simulink model "NN_v01"  (R2018b)
settings: Solver=VariableStepAuto  StartTime=0.0  StopTime=10.0  RelTol=1e-3
values from neighbouring files (symbols this model uses):
  B = 0.5    [Matlab_Newton_simulation_v01.m]    (also in NewtonMethod.m; NewtonMethod_2.m = 0.3; System_parameters.m = 0.3)
  b = f    (= 0.01)    [Matlab_Newton_simulation_v01.m]    (also in NewtonMethod.m; System_parameters.m)
  in_NN_data = [0 -100 -100 -100 -100 -100 -100 -100 -100 -100 -100 -100 ... (160801 elements, 401x401)]    [NN_IO_data.mat]    (also in NN_generate_input_data.m = con2seq(in_NN_data); NN_modelling_v02.m = con2seq(in_NN_data); NN_modelling_v03.m = con2seq(in_NN_data))
  l = 0.1    [Matlab_Newton_simulation_v01.m]    (also in NewtonMethod.m; NewtonMethod_2.m; System_parameters.m)
  m = 0.04    [Matlab_Newton_simulation_v01.m]    (also in NewtonMethod.m = 0.1; NewtonMethod_2.m; System_parameters.m)
  R = 1    [Matlab_Newton_simulation_v01.m]    (also in NewtonMethod.m; NewtonMethod_2.m = 0.1; System_parameters.m = 0.1)
libraries: neural x128
(part 5 of 5)

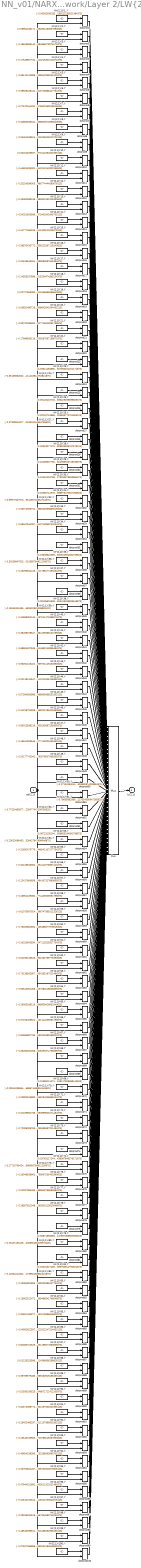
== system NN_v01/NARX Neural Network/Layer 2/LW{2,1} ==
  "ad{2,1}" : Inport  PortDimensions=10  SampleTime=1
      mask Display: e = 0.06;c1 = [120 230 180]/255;c2 = ([120 230 180]+0)/(256+128);c3 = ([120 230 180]+128)/(256+128);patch([0 1 1 0],[0 0 1 1],c1);patch([0 1 1 1-e 1-e 0+e],[0 0 1 1-e 0+e 0+e],c2);patch([0 0 1 1-e 0+e 0+e],[0 1 1 1-e 1-e 0+e],c3);plot([0 1 1 0 0],[0 0 1 1 0]);
  "IW{2,1}(1,:)'" : Constant  Value=[-0.00582930285020249842886652658080492983572185039520263671875;0.341294044267576091034044338812236674129962921142578125;0.275034396637413081077028209620038978755474090576171875;0.2474633161173106221664141912697232328355312347412109375;-1.50248270345251366819638860761187970638275146484375;0.7732400327116855098807945978478528559207916259765625;-0.463470385585337485423451653332449495792388916015625;-1.78313893365298614668290611007250845432281494140625;-0.8519246471113970375910184884560294449329376220703125;1.011244644169964512769865905283950269222259521484375]
      mask Display: e = 0.06;c1 = [120 150 230]/255;c2 = ([120 150 230]+0)/383;c3 = ([120 150 230]+128)/383;patch([0 1 1 0],[0 0 1 1],c1);patch([0 1 1 1-e 1-e 0+e],[0 0 1 1-e 0+e 0+e],c2);patch([0 0 1 1-e 0+e 0+e],[0 1 1 1-e 1-e 0+e],c3);plot([0 1 1 0 0],[0 0 1 1 0]);disp('weights');
  "IW{2,1}(10,:)'" : Constant  Value=[0.0020462983754603873871869001987988667679019272327423095703125;0.56448793796692864344066720150294713675975799560546875;1.50097031622448895404886570759117603302001953125;-0.43999986998791829062582792175817303359508514404296875;-2.436220494401638791970299280364997684955596923828125;0.90173545642475871897403294497053138911724090576171875;0.20243963357671435066009735237457789480686187744140625;0.359896850926928524305736800670274533331394195556640625;-0.9562162738582724585967298480682075023651123046875;1.2001988168349815300217642288771457970142364501953125]
      mask Display: e = 0.06;c1 = [120 150 230]/255;c2 = ([120 150 230]+0)/383;c3 = ([120 150 230]+128)/383;patch([0 1 1 0],[0 0 1 1],c1);patch([0 1 1 1-e 1-e 0+e],[0 0 1 1-e 0+e 0+e],c2);patch([0 0 1 1-e 0+e 0+e],[0 1 1 1-e 1-e 0+e],c3);plot([0 1 1 0 0],[0 0 1 1 0]);disp('weights');
  "IW{2,1}(100,:)'" : Constant  Value=[-0.07507286886552631821611925033721490763127803802490234375;0.59504324954741238951072546115028671920299530029296875;1.5961364935602364578670631090062670409679412841796875;-0.49363437154612432866684912369237281382083892822265625;-2.671162470519930831613919508527033030986785888671875;1.0123483498732077645598792514647357165813446044921875;0.236650285271016669330634840662241913378238677978515625;0.1698534154758429559617383119984879158437252044677734375;-1.2007351974579927311737037598504684865474700927734375;0.426723506364093230214251661891466937959194183349609375]
      mask Display: e = 0.06;c1 = [120 150 230]/255;c2 = ([120 150 230]+0)/383;c3 = ([120 150 230]+128)/383;patch([0 1 1 0],[0 0 1 1],c1);patch([0 1 1 1-e 1-e 0+e],[0 0 1 1-e 0+e 0+e],c2);patch([0 0 1 1-e 0+e 0+e],[0 1 1 1-e 1-e 0+e],c3);plot([0 1 1 0 0],[0 0 1 1 0]);disp('weights');
  "IW{2,1}(11,:)'" : Constant  Value=[-0.448513060024906928813237527720048092305660247802734375;0.64031830164589853549017561817890964448451995849609375;2.099861680687876486217646743170917034149169921875;-0.407344506580868459533206760170287452638149261474609375;-1.4883679183223523789791897797840647399425506591796875;1.4010738816362786618441305108717642724514007568359375;0.09498188052392357583197934900454129092395305633544921875;0.11685031296741331396926710795014514587819576263427734375;-1.1492554861913626407243782523437403142452239990234375;1.1105840548960890235008491799817420542240142822265625]
      mask Display: e = 0.06;c1 = [120 150 230]/255;c2 = ([120 150 230]+0)/383;c3 = ([120 150 230]+128)/383;patch([0 1 1 0],[0 0 1 1],c1);patch([0 1 1 1-e 1-e 0+e],[0 0 1 1-e 0+e 0+e],c2);patch([0 0 1 1-e 0+e 0+e],[0 1 1 1-e 1-e 0+e],c3);plot([0 1 1 0 0],[0 0 1 1 0]);disp('weights');
  "IW{2,1}(12,:)'" : Constant  Value=[-0.323245990037860642107858666349784471094608306884765625;0.702947047886376186198731375043280422687530517578125;2.15919372922789865043569079716689884662628173828125;-0.1613313202849812333372625516858533956110477447509765625;-2.691776450442475709934342376072891056537628173828125;1.3935502725959150183143719914369285106658935546875;-0.156722502399286034435732517522410489618778228759765625;-0.546597317678598759727037759148515760898590087890625;-0.0575394611420758927966545570598100312054157257080078125;0.2566683614467841767492473081802017986774444580078125]
      mask Display: e = 0.06;c1 = [120 150 230]/255;c2 = ([120 150 230]+0)/383;c3 = ([120 150 230]+128)/383;patch([0 1 1 0],[0 0 1 1],c1);patch([0 1 1 1-e 1-e 0+e],[0 0 1 1-e 0+e 0+e],c2);patch([0 0 1 1-e 0+e 0+e],[0 1 1 1-e 1-e 0+e],c3);plot([0 1 1 0 0],[0 0 1 1 0]);disp('weights');
  "IW{2,1}(13,:)'" : Constant  Value=[-0.45062389136594493965759511411306448280811309814453125;0.74707514561312782230828588581061922013759613037109375;2.534602836838535377950165639049373567104339599609375;0.681856533543756082593745304620824754238128662109375;-1.903748935623813309803153970278799533843994140625;1.486962257730305214664667801116593182086944580078125;-0.97748822795309264765961643206537701189517974853515625;-0.66163025511440742842950157864834181964397430419921875;-0.2757918190568944272200724299182184040546417236328125;0.3709896375713379601535280016832984983921051025390625]
      mask Display: e = 0.06;c1 = [120 150 230]/255;c2 = ([120 150 230]+0)/383;c3 = ([120 150 230]+128)/383;patch([0 1 1 0],[0 0 1 1],c1);patch([0 1 1 1-e 1-e 0+e],[0 0 1 1-e 0+e 0+e],c2);patch([0 0 1 1-e 0+e 0+e],[0 1 1 1-e 1-e 0+e],c3);plot([0 1 1 0 0],[0 0 1 1 0]);disp('weights');
  "IW{2,1}(14,:)'" : Constant  Value=[-0.54251603589707408925590925719006918370723724365234375;0.66743961741495472228535845715668983757495880126953125;2.25752081983530050734998440020717680454254150390625;-0.5193854735052190196853416637168265879154205322265625;-0.9760728597570194065013993167667649686336517333984375;1.5237519361875244694459752281545661389827728271484375;0.18414734508753072272924100616364739835262298583984375;-0.51378704789147111586800065197166986763477325439453125;-1.460284612501698386921589190023951232433319091796875;0.5274995341412360705390938164782710373401641845703125]
      mask Display: e = 0.06;c1 = [120 150 230]/255;c2 = ([120 150 230]+0)/383;c3 = ([120 150 230]+128)/383;patch([0 1 1 0],[0 0 1 1],c1);patch([0 1 1 1-e 1-e 0+e],[0 0 1 1-e 0+e 0+e],c2);patch([0 0 1 1-e 0+e 0+e],[0 1 1 1-e 1-e 0+e],c3);plot([0 1 1 0 0],[0 0 1 1 0]);disp('weights');
  "IW{2,1}(15,:)'" : Constant  Value=[-0.447774651064073492268136078564566560089588165283203125;0.791075818282777287748785965959541499614715576171875;2.658332437781770973828088244772516191005706787109375;0.19098785388139061236500992890796624124050140380859375;-2.357140652927365298552331296377815306186676025390625;1.6002796151954721270982417991035617887973785400390625;-0.533911807011674621747943092486821115016937255859375;-1.139783609828504129524162635789252817630767822265625;0.64540001022538107111614635869045741856098175048828125;0.231918187426728927835739568763528950512409210205078125]
      mask Display: e = 0.06;c1 = [120 150 230]/255;c2 = ([120 150 230]+0)/383;c3 = ([120 150 230]+128)/383;patch([0 1 1 0],[0 0 1 1],c1);patch([0 1 1 1-e 1-e 0+e],[0 0 1 1-e 0+e 0+e],c2);patch([0 0 1 1-e 0+e 0+e],[0 1 1 1-e 1-e 0+e],c3);plot([0 1 1 0 0],[0 0 1 1 0]);disp('weights');
  "IW{2,1}(16,:)'" : Constant  Value=[-0.368704337726813380360368910260149277746677398681640625;0.71983605028876151976646724506281316280364990234375;2.34431403126588211449643495143391191959381103515625;-0.284742382385777925701830781690659932792186737060546875;-2.320518919797865731169395075994543731212615966796875;1.45456918782064992257119229179807007312774658203125;-0.046608776255616470030052056472413823939859867095947265625;-0.44794291876033776045318290925933979451656341552734375;0.26754547078348134281355896746390499174594879150390625;0.8955736134500613676578950617113150656223297119140625]
      mask Display: e = 0.06;c1 = [120 150 230]/255;c2 = ([120 150 230]+0)/383;c3 = ([120 150 230]+128)/383;patch([0 1 1 0],[0 0 1 1],c1);patch([0 1 1 1-e 1-e 0+e],[0 0 1 1-e 0+e 0+e],c2);patch([0 0 1 1-e 0+e 0+e],[0 1 1 1-e 1-e 0+e],c3);plot([0 1 1 0 0],[0 0 1 1 0]);disp('weights');
  "IW{2,1}(17,:)'" : Constant  Value=[-0.316196432043710562442839773211744613945484161376953125;0.65170561350326738914162660876172594726085662841796875;2.052447913065332141258068077149800956249237060546875;0.1414451597873920551950988055978086777031421661376953125;-1.656287054632532118603194248862564563751220703125;1.2539456102076791399468902454827912151813507080078125;-0.41024093016196083727464838375453837215900421142578125;-0.305332211388109342475871699207345955073833465576171875;-1.38320146192491666425894436542876064777374267578125;0.34265345297769600474424578351317904889583587646484375]
      mask Display: e = 0.06;c1 = [120 150 230]/255;c2 = ([120 150 230]+0)/383;c3 = ([120 150 230]+128)/383;patch([0 1 1 0],[0 0 1 1],c1);patch([0 1 1 1-e 1-e 0+e],[0 0 1 1-e 0+e 0+e],c2);patch([0 0 1 1-e 0+e 0+e],[0 1 1 1-e 1-e 0+e],c3);plot([0 1 1 0 0],[0 0 1 1 0]);disp('weights');
  "IW{2,1}(18,:)'" : Constant  Value=[-0.1455533789674021971638495642764610238373279571533203125;0.6124068528724364579574057643185369670391082763671875;1.8468413066792230825541309968684799969196319580078125;0.2195780819216167356611180139225325547158718109130859375;-1.5780996737606607371873224110458977520465850830078125;1.0438697054205532399606681792647577822208404541015625;-0.452505406111580354977519391468376852571964263916015625;-0.257559752512215578423848683087271638214588165283203125;-1.2582096901281809575579018201096914708614349365234375;0.8091801339623978517323621417745016515254974365234375]
      mask Display: e = 0.06;c1 = [120 150 230]/255;c2 = ([120 150 230]+0)/383;c3 = ([120 150 230]+128)/383;patch([0 1 1 0],[0 0 1 1],c1);patch([0 1 1 1-e 1-e 0+e],[0 0 1 1-e 0+e 0+e],c2);patch([0 0 1 1-e 0+e 0+e],[0 1 1 1-e 1-e 0+e],c3);plot([0 1 1 0 0],[0 0 1 1 0]);disp('weights');
  "IW{2,1}(19,:)'" : Constant  Value=[0.0272765608292123602762746514827085775323212146759033203125;0.60751700312979561857673616032116115093231201171875;1.5496728878781473870418494698242284357547760009765625;-0.2376857676320399959113416343825520016252994537353515625;-3.088549185031914223742433023289777338504791259765625;0.92990955504973638046095629761111922562122344970703125;-0.00135475849347249720049102261754114806535653769969940185546875;-0.10569070740692888821232742202482768334448337554931640625;-0.959228755518120035361562258913181722164154052734375;0.017495673838348692330502132108449586667120456695556640625]
      mask Display: e = 0.06;c1 = [120 150 230]/255;c2 = ([120 150 230]+0)/383;c3 = ([120 150 230]+128)/383;patch([0 1 1 0],[0 0 1 1],c1);patch([0 1 1 1-e 1-e 0+e],[0 0 1 1-e 0+e 0+e],c2);patch([0 0 1 1-e 0+e 0+e],[0 1 1 1-e 1-e 0+e],c3);plot([0 1 1 0 0],[0 0 1 1 0]);disp('weights');
  "IW{2,1}(2,:)'" : Constant  Value=[0.05954166171467280277429523493992746807634830474853515625;0.40883309461008676688464902326813898980617523193359375;0.54706995308614458917162437501247040927410125732421875;-0.70577749899209096806629304410307668149471282958984375;-2.0501531346926782362061203457415103912353515625;0.79578752445065259468748308790964074432849884033203125;0.455298404531613964962843965622596442699432373046875;-1.261341483048185718729428117512725293636322021484375;-1.3307058361577859262325773670454509556293487548828125;0.351381921406758834791617118753492832183837890625]
      mask Display: e = 0.06;c1 = [120 150 230]/255;c2 = ([120 150 230]+0)/383;c3 = ([120 150 230]+128)/383;patch([0 1 1 0],[0 0 1 1],c1);patch([0 1 1 1-e 1-e 0+e],[0 0 1 1-e 0+e 0+e],c2);patch([0 0 1 1-e 0+e 0+e],[0 1 1 1-e 1-e 0+e],c3);plot([0 1 1 0 0],[0 0 1 1 0]);disp('weights');
  "IW{2,1}(20,:)'" : Constant  Value=[-0.038314807160081378045735078785583027638494968414306640625;0.64192842298741126239036702827434055507183074951171875;1.7730670440839084722739471544628031551837921142578125;-0.2070422965789282254700509611211600713431835174560546875;-2.049795488218523420442807037034071981906890869140625;1.05160185870840994226682596490718424320220947265625;-0.056829012384008115166267316453740932047367095947265625;-1.4674161260953708652010618607164360582828521728515625;-0.713738154031241744945646132691763341426849365234375;-0.280871218212835505045887884989497251808643341064453125]
      mask Display: e = 0.06;c1 = [120 150 230]/255;c2 = ([120 150 230]+0)/383;c3 = ([120 150 230]+128)/383;patch([0 1 1 0],[0 0 1 1],c1);patch([0 1 1 1-e 1-e 0+e],[0 0 1 1-e 0+e 0+e],c2);patch([0 0 1 1-e 0+e 0+e],[0 1 1 1-e 1-e 0+e],c3);plot([0 1 1 0 0],[0 0 1 1 0]);disp('weights');
  "IW{2,1}(21,:)'" : Constant  Value=[-0.59732069362601347695118647607159800827503204345703125;0.7944289114524234474146169304731301963329315185546875;2.771254282326547357939716675900854170322418212890625;-0.2278187864269799189909093684036633931100368499755859375;-2.350390468410268329790824282099492847919464111328125;1.769409008533941563001690155942924320697784423828125;-0.156797325798515074790628887058119289577007293701171875;-0.6081986540006287800252948727575130760669708251953125;0.9005540148021478064066513979923911392688751220703125;0.908050065992017874094699436682276427745819091796875]
      mask Display: e = 0.06;c1 = [120 150 230]/255;c2 = ([120 150 230]+0)/383;c3 = ([120 150 230]+128)/383;patch([0 1 1 0],[0 0 1 1],c1);patch([0 1 1 1-e 1-e 0+e],[0 0 1 1-e 0+e 0+e],c2);patch([0 0 1 1-e 0+e 0+e],[0 1 1 1-e 1-e 0+e],c3);plot([0 1 1 0 0],[0 0 1 1 0]);disp('weights');
  "IW{2,1}(22,:)'" : Constant  Value=[-0.1799665611847947044310558339930139482021331787109375;0.597358676332699456423824813100509345531463623046875;1.7143661042907727409811968755093403160572052001953125;-0.73930354885972360268198144694906659424304962158203125;-1.4961714010009259379074819662491790950298309326171875;1.122458137878769690587432705797255039215087890625;0.457656457228035329354298710313742049038410186767578125;-0.669106619974649152737811164115555584430694580078125;-1.6311188924677946232577596674673259258270263671875;0.219954413074346433187855609503458254039287567138671875]
      mask Display: e = 0.06;c1 = [120 150 230]/255;c2 = ([120 150 230]+0)/383;c3 = ([120 150 230]+128)/383;patch([0 1 1 0],[0 0 1 1],c1);patch([0 1 1 1-e 1-e 0+e],[0 0 1 1-e 0+e 0+e],c2);patch([0 0 1 1-e 0+e 0+e],[0 1 1 1-e 1-e 0+e],c3);plot([0 1 1 0 0],[0 0 1 1 0]);disp('weights');
  "IW{2,1}(23,:)'" : Constant  Value=[0.03514453865765392037712189221565495245158672332763671875;0.583844705291804100255603771074675023555755615234375;1.486426002621094699662762650405056774616241455078125;-0.90210579101266075152665280256769619882106781005859375;-2.997563508188325176462285526213236153125762939453125;0.94298906502310886335038730976521037518978118896484375;0.6341705941798434498224423805368132889270782470703125;0.1574250096667909326608736364505602978169918060302734375;-0.4923218586946191965836305826087482273578643798828125;0.90542674776050702245555612535099498927593231201171875]
      mask Display: e = 0.06;c1 = [120 150 230]/255;c2 = ([120 150 230]+0)/383;c3 = ([120 150 230]+128)/383;patch([0 1 1 0],[0 0 1 1],c1);patch([0 1 1 1-e 1-e 0+e],[0 0 1 1-e 0+e 0+e],c2);patch([0 0 1 1-e 0+e 0+e],[0 1 1 1-e 1-e 0+e],c3);plot([0 1 1 0 0],[0 0 1 1 0]);disp('weights');
  "IW{2,1}(24,:)'" : Constant  Value=[-0.35136664502954972899573249378590844571590423583984375;0.6736465513516909364710727459168992936611175537109375;2.144522192177507946553305373527109622955322265625;-0.5348072314147584993548889542580582201480865478515625;-1.8134291528864909803786531483638100326061248779296875;1.38047161618545288774839718826115131378173828125;0.21260601550874402843049892908311448991298675537109375;-0.5304234087346137993534966881270520389080047607421875;-0.574433193811335396361528182751499116420745849609375;0.67345838441960104159278444058145396411418914794921875]
      mask Display: e = 0.06;c1 = [120 150 230]/255;c2 = ([120 150 230]+0)/383;c3 = ([120 150 230]+128)/383;patch([0 1 1 0],[0 0 1 1],c1);patch([0 1 1 1-e 1-e 0+e],[0 0 1 1-e 0+e 0+e],c2);patch([0 0 1 1-e 0+e 0+e],[0 1 1 1-e 1-e 0+e],c3);plot([0 1 1 0 0],[0 0 1 1 0]);disp('weights');
  "IW{2,1}(25,:)'" : Constant  Value=[0.05149415733482787249641887683537788689136505126953125;0.55009804320874489125259287902736105024814605712890625;1.4573734074988748954382344891200773417949676513671875;0.203985369914554570680564893336850218474864959716796875;-2.108439519484554214301397223607636988162994384765625;0.7713724398957200190096727965283207595348358154296875;-0.38913427522632348942721591811277903616428375244140625;0.40356097259732670590182124215061776340007781982421875;-1.686695031530128563446169209782965481281280517578125;0.89980821268971344917275700936443172395229339599609375]
      mask Display: e = 0.06;c1 = [120 150 230]/255;c2 = ([120 150 230]+0)/383;c3 = ([120 150 230]+128)/383;patch([0 1 1 0],[0 0 1 1],c1);patch([0 1 1 1-e 1-e 0+e],[0 0 1 1-e 0+e 0+e],c2);patch([0 0 1 1-e 0+e 0+e],[0 1 1 1-e 1-e 0+e],c3);plot([0 1 1 0 0],[0 0 1 1 0]);disp('weights');
  "IW{2,1}(26,:)'" : Constant  Value=[0.02204713886760389929264647435047663748264312744140625;0.5921585247554281838944234550581313669681549072265625;1.55519918105156396137545016244985163211822509765625;-0.51973881437109403780283400919870473444461822509765625;-2.912447784998210220663850122946314513683319091796875;0.93575628387550702225183840710087679326534271240234375;0.268635001612249457725312140610185451805591583251953125;0.2139320565909990923270100893205380998551845550537109375;-0.5458971643579728638684400721103884279727935791015625;0.93073309088335609562392392035690136253833770751953125]
      mask Display: e = 0.06;c1 = [120 150 230]/255;c2 = ([120 150 230]+0)/383;c3 = ([120 150 230]+128)/383;patch([0 1 1 0],[0 0 1 1],c1);patch([0 1 1 1-e 1-e 0+e],[0 0 1 1-e 0+e 0+e],c2);patch([0 0 1 1-e 0+e 0+e],[0 1 1 1-e 1-e 0+e],c3);plot([0 1 1 0 0],[0 0 1 1 0]);disp('weights');
  "IW{2,1}(27,:)'" : Constant  Value=[-0.37908624877066599001551594483316875994205474853515625;0.7418677921218022053295726436772383749485015869140625;2.443837843676642140877675046795047819614410400390625;-0.02623926447862567901125885327928699553012847900390625;-2.2303123439129013405590740148909389972686767578125;1.4856482550534242381701233171042986214160919189453125;-0.303941770708726632932439315482042729854583740234375;-0.82184113198571473457576530563528649508953094482421875;0.485827492873038779830352495991974137723445892333984375;0.72913166625223502226305072326795198023319244384765625]
      mask Display: e = 0.06;c1 = [120 150 230]/255;c2 = ([120 150 230]+0)/383;c3 = ([120 150 230]+128)/383;patch([0 1 1 0],[0 0 1 1],c1);patch([0 1 1 1-e 1-e 0+e],[0 0 1 1-e 0+e 0+e],c2);patch([0 0 1 1-e 0+e 0+e],[0 1 1 1-e 1-e 0+e],c3);plot([0 1 1 0 0],[0 0 1 1 0]);disp('weights');
  "IW{2,1}(28,:)'" : Constant  Value=[0.0262307747004455575623449448130486416630446910858154296875;0.6141526444488019098599806966376490890979766845703125;1.68407366789876089541166948038153350353240966796875;0.396007677131411828241880357381887733936309814453125;-2.224396987240094603066609124653041362762451171875;0.89300425378741821180739179908414371311664581298828125;-0.6041927337275698750573837969568558037281036376953125;-0.586160540594302670314164060982875525951385498046875;-1.0496445142758663582327471885946579277515411376953125;0.1955911512259201068264502509919111616909503936767578125]
      mask Display: e = 0.06;c1 = [120 150 230]/255;c2 = ([120 150 230]+0)/383;c3 = ([120 150 230]+128)/383;patch([0 1 1 0],[0 0 1 1],c1);patch([0 1 1 1-e 1-e 0+e],[0 0 1 1-e 0+e 0+e],c2);patch([0 0 1 1-e 0+e 0+e],[0 1 1 1-e 1-e 0+e],c3);plot([0 1 1 0 0],[0 0 1 1 0]);disp('weights');
  "IW{2,1}(29,:)'" : Constant  Value=[0.0246853775513488395143557596611572080291807651519775390625;0.57664087857391665981054984513320960104465484619140625;1.519319484599648273359662198345176875591278076171875;-0.414640620269337734082881752328830771148204803466796875;-2.36036201032834380697522647096775472164154052734375;0.8965136872108658838698147519608028233051300048828125;0.177479815810386798435871469337143935263156890869140625;-0.0696335087218894199789787080590031109750270843505859375;-1.038098982722849061843817253247834742069244384765625;0.74747558926703472348407331082853488624095916748046875]
      mask Display: e = 0.06;c1 = [120 150 230]/255;c2 = ([120 150 230]+0)/383;c3 = ([120 150 230]+128)/383;patch([0 1 1 0],[0 0 1 1],c1);patch([0 1 1 1-e 1-e 0+e],[0 0 1 1-e 0+e 0+e],c2);patch([0 0 1 1-e 0+e 0+e],[0 1 1 1-e 1-e 0+e],c3);plot([0 1 1 0 0],[0 0 1 1 0]);disp('weights');
  "IW{2,1}(3,:)'" : Constant  Value=[-0.1684585614083785320982400435241288505494594573974609375;0.48589007836087583225292974020703695714473724365234375;1.1686058202574383102501087705604732036590576171875;-0.0581777076386999769663788129037129692733287811279296875;-1.262969470679580208383185890852473676204681396484375;1.009868185502584392310154726146720349788665771484375;-0.191550045020977333098954886736464686691761016845703125;-0.8789087611980193059935118071734905242919921875;-1.4777892930254401537837338764802552759647369384765625;0.82183474981515203250381773614208213984966278076171875]
      mask Display: e = 0.06;c1 = [120 150 230]/255;c2 = ([120 150 230]+0)/383;c3 = ([120 150 230]+128)/383;patch([0 1 1 0],[0 0 1 1],c1);patch([0 1 1 1-e 1-e 0+e],[0 0 1 1-e 0+e 0+e],c2);patch([0 0 1 1-e 0+e 0+e],[0 1 1 1-e 1-e 0+e],c3);plot([0 1 1 0 0],[0 0 1 1 0]);disp('weights');
  "IW{2,1}(30,:)'" : Constant  Value=[0.1525421876865361292541223292573704384267330169677734375;0.59280217846434168915692453083465807139873504638671875;1.5103998560570150999637917266227304935455322265625;0.6179532744324938153823723041568882763385772705078125;-2.27436947201279071606450088438577950000762939453125;0.73383641375792552086210207562544383108615875244140625;-0.79185101288714199174734176267520524561405181884765625;-0.78250730160382298006283008362515829503536224365234375;-1.3421010523912026979331812981399707496166229248046875;-0.170860963215741123999436013036756776273250579833984375]
      mask Display: e = 0.06;c1 = [120 150 230]/255;c2 = ([120 150 230]+0)/383;c3 = ([120 150 230]+128)/383;patch([0 1 1 0],[0 0 1 1],c1);patch([0 1 1 1-e 1-e 0+e],[0 0 1 1-e 0+e 0+e],c2);patch([0 0 1 1-e 0+e 0+e],[0 1 1 1-e 1-e 0+e],c3);plot([0 1 1 0 0],[0 0 1 1 0]);disp('weights');
  "IW{2,1}(31,:)'" : Constant  Value=[0.25380712576948349923355863211327232420444488525390625;0.492216462292187573179802484446554444730281829833984375;0.99693922666631429319039625625009648501873016357421875;-0.49533921863121566087073688322561793029308319091796875;-2.790527644025747378009327803738415241241455078125;0.56383871163692311778703469826723448932170867919921875;0.31609849703952985766619576679659076035022735595703125;0.50949914899270487556037778631434775888919830322265625;-1.9496983918952286440884336116141639649868011474609375;0.50011526375033188429597430513240396976470947265625]
      mask Display: e = 0.06;c1 = [120 150 230]/255;c2 = ([120 150 230]+0)/383;c3 = ([120 150 230]+128)/383;patch([0 1 1 0],[0 0 1 1],c1);patch([0 1 1 1-e 1-e 0+e],[0 0 1 1-e 0+e 0+e],c2);patch([0 0 1 1-e 0+e 0+e],[0 1 1 1-e 1-e 0+e],c3);plot([0 1 1 0 0],[0 0 1 1 0]);disp('weights');
  "IW{2,1}(32,:)'" : Constant  Value=[-0.59977927573484135503889547180733643472194671630859375;0.78607459639563870279488355663488619029521942138671875;2.72389386341507577782294902135618031024932861328125;-0.373262242287550394248540897024213336408138275146484375;-2.49918566630663452343696917523629963397979736328125;1.77057144387650833294856056454591453075408935546875;-0.0165541406353492855096920521873471443541347980499267578125;-0.40925534192587742499114256133907474577426910400390625;0.8975452209878096443418371563893742859363555908203125;0.9980060058792241672875888980343006551265716552734375]
      mask Display: e = 0.06;c1 = [120 150 230]/255;c2 = ([120 150 230]+0)/383;c3 = ([120 150 230]+128)/383;patch([0 1 1 0],[0 0 1 1],c1);patch([0 1 1 1-e 1-e 0+e],[0 0 1 1-e 0+e 0+e],c2);patch([0 0 1 1-e 0+e 0+e],[0 1 1 1-e 1-e 0+e],c3);plot([0 1 1 0 0],[0 0 1 1 0]);disp('weights');
  "IW{2,1}(33,:)'" : Constant  Value=[-0.05374356701386216739191326041691354475915431976318359375;0.60138254176158145725139547721482813358306884765625;1.599503658211905321451240524766035377979278564453125;-0.8636852631541216407384808917413465678691864013671875;-2.845568136452600871422191630699671804904937744140625;1.0405825744174703739730603047064505517482757568359375;0.58290688850284488875530541918124072253704071044921875;0.051528965566472302584077880283075501210987567901611328125;-0.66103580577425147257741855355561710894107818603515625;0.66779080122559675292137626456678844988346099853515625]
      mask Display: e = 0.06;c1 = [120 150 230]/255;c2 = ([120 150 230]+0)/383;c3 = ([120 150 230]+128)/383;patch([0 1 1 0],[0 0 1 1],c1);patch([0 1 1 1-e 1-e 0+e],[0 0 1 1-e 0+e 0+e],c2);patch([0 0 1 1-e 0+e 0+e],[0 1 1 1-e 1-e 0+e],c3);plot([0 1 1 0 0],[0 0 1 1 0]);disp('weights');
  "IW{2,1}(34,:)'" : Constant  Value=[-0.581678440979031652346975533873774111270904541015625;0.81326669444152577259643521756515838205814361572265625;2.89315911107999834683823792147450149059295654296875;0.70491023718167389322530880235717631876468658447265625;-2.18278968945419915570482771727256476879119873046875;1.7147670503171494882366232559434138238430023193359375;-1.045237944023320597608517346088774502277374267578125;-0.70802493541687494538194869164726696908473968505859375;0.880677613510830070708834682591259479522705078125;0.84463766908679482892097212243243120610713958740234375]
      mask Display: e = 0.06;c1 = [120 150 230]/255;c2 = ([120 150 230]+0)/383;c3 = ([120 150 230]+128)/383;patch([0 1 1 0],[0 0 1 1],c1);patch([0 1 1 1-e 1-e 0+e],[0 0 1 1-e 0+e 0+e],c2);patch([0 0 1 1-e 0+e 0+e],[0 1 1 1-e 1-e 0+e],c3);plot([0 1 1 0 0],[0 0 1 1 0]);disp('weights');
  "IW{2,1}(35,:)'" : Constant  Value=[0.196066220897142706736104855735902674496173858642578125;0.56114967567245077617599235964007675647735595703125;1.3132272740157155954676682085846550762653350830078125;-0.190190351808331492566850329239969141781330108642578125;-3.4050286399046942875656895921565592288970947265625;0.711621044678856673471045723999850451946258544921875;-0.01169746299349863453975739702173086698167026042938232421875;0.53162953097797494006471197280916385352611541748046875;-0.6906821766335207168907572850002907216548919677734375;0.8527130315578423935818364043370820581912994384765625]
      mask Display: e = 0.06;c1 = [120 150 230]/255;c2 = ([120 150 230]+0)/383;c3 = ([120 150 230]+128)/383;patch([0 1 1 0],[0 0 1 1],c1);patch([0 1 1 1-e 1-e 0+e],[0 0 1 1-e 0+e 0+e],c2);patch([0 0 1 1-e 0+e 0+e],[0 1 1 1-e 1-e 0+e],c3);plot([0 1 1 0 0],[0 0 1 1 0]);disp('weights');
  "IW{2,1}(36,:)'" : Constant  Value=[-0.30238847823709935624947320320643484592437744140625;0.63809581334946396946605773337068967521190643310546875;1.93841310136525013518848936655558645725250244140625;-0.76799610669453122202554595787660218775272369384765625;-1.790601099870265944247194056515581905841827392578125;1.2946912691900547276446786781889386475086212158203125;0.455166148167682471648021191867883317172527313232421875;-0.449030326835419713038533018334419466555118560791015625;-1.1676394023242508968252195700188167393207550048828125;0.383807058733641459635776982395327650010585784912109375]
      mask Display: e = 0.06;c1 = [120 150 230]/255;c2 = ([120 150 230]+0)/383;c3 = ([120 150 230]+128)/383;patch([0 1 1 0],[0 0 1 1],c1);patch([0 1 1 1-e 1-e 0+e],[0 0 1 1-e 0+e 0+e],c2);patch([0 0 1 1-e 0+e 0+e],[0 1 1 1-e 1-e 0+e],c3);plot([0 1 1 0 0],[0 0 1 1 0]);disp('weights');
  "IW{2,1}(37,:)'" : Constant  Value=[-0.452936344163830550968441457371227443218231201171875;0.76433820653682549295382386844721622765064239501953125;2.56830362490622832183362334035336971282958984375;0.5183817105699082272707300944603048264980316162109375;-1.8382729426133825878508787354803644120693206787109375;1.5372946831195355432697624564752914011478424072265625;-0.83324123394107785234297125498414970934391021728515625;-1.2789096058712516867927888597478158771991729736328125;-0.106021597656944133181156075806939043104648590087890625;-0.054355271524427505036580754449460073374211788177490234375]
      mask Display: e = 0.06;c1 = [120 150 230]/255;c2 = ([120 150 230]+0)/383;c3 = ([120 150 230]+128)/383;patch([0 1 1 0],[0 0 1 1],c1);patch([0 1 1 1-e 1-e 0+e],[0 0 1 1-e 0+e 0+e],c2);patch([0 0 1 1-e 0+e 0+e],[0 1 1 1-e 1-e 0+e],c3);plot([0 1 1 0 0],[0 0 1 1 0]);disp('weights');
  "IW{2,1}(38,:)'" : Constant  Value=[0.09136601508625417922271338966311304830014705657958984375;0.62253057715237625213688943404122255742549896240234375;1.627047130871312585753685198142193257808685302734375;0.176907776487810475263273701784783042967319488525390625;-2.82675092583253739775273061241023242473602294921875;0.87596723158291622812754440019489265978336334228515625;-0.396760044760268326680119344018748961389064788818359375;-0.60181119810399430480885030192439444363117218017578125;-0.53741128759564638084356147373910062015056610107421875;0.1372008230337089240702397319182637147605419158935546875]
      mask Display: e = 0.06;c1 = [120 150 230]/255;c2 = ([120 150 230]+0)/383;c3 = ([120 150 230]+128)/383;patch([0 1 1 0],[0 0 1 1],c1);patch([0 1 1 1-e 1-e 0+e],[0 0 1 1-e 0+e 0+e],c2);patch([0 0 1 1-e 0+e 0+e],[0 1 1 1-e 1-e 0+e],c3);plot([0 1 1 0 0],[0 0 1 1 0]);disp('weights');
  "IW{2,1}(39,:)'" : Constant  Value=[-0.1834530433555252304511640204509603790938854217529296875;0.59972841849818703252594787045381963253021240234375;1.80972193123266134051618792000226676464080810546875;-0.214511595761017748174026564811356365680694580078125;-1.818294281749900154210308755864389240741729736328125;1.0839633537532911145007119557703845202922821044921875;-0.038703040293351233247509668444763519801199436187744140625;0.31497073227985061816269762857700698077678680419921875;-1.217905982251902496926732055726461112499237060546875;1.219166080770367699415146489627659320831298828125]
      mask Display: e = 0.06;c1 = [120 150 230]/255;c2 = ([120 150 230]+0)/383;c3 = ([120 150 230]+128)/383;patch([0 1 1 0],[0 0 1 1],c1);patch([0 1 1 1-e 1-e 0+e],[0 0 1 1-e 0+e 0+e],c2);patch([0 0 1 1-e 0+e 0+e],[0 1 1 1-e 1-e 0+e],c3);plot([0 1 1 0 0],[0 0 1 1 0]);disp('weights');
  "IW{2,1}(4,:)'" : Constant  Value=[-0.1764985773415378711437284664498292841017246246337890625;0.550065938829558565004163028788752853870391845703125;1.400052168430072629945470907841809093952178955078125;0.132046705074750747588296917456318624317646026611328125;-1.7551038520745418924917657932383008301258087158203125;1.1042013956640885918858430159161798655986785888671875;-0.398070213018517471414980946065043099224567413330078125;-1.2779459978482663462528989839483983814716339111328125;-0.74348434077020153498693844085210002958774566650390625;0.43747499192806316159476409666240215301513671875]
      mask Display: e = 0.06;c1 = [120 150 230]/255;c2 = ([120 150 230]+0)/383;c3 = ([120 150 230]+128)/383;patch([0 1 1 0],[0 0 1 1],c1);patch([0 1 1 1-e 1-e 0+e],[0 0 1 1-e 0+e 0+e],c2);patch([0 0 1 1-e 0+e 0+e],[0 1 1 1-e 1-e 0+e],c3);plot([0 1 1 0 0],[0 0 1 1 0]);disp('weights');
  "IW{2,1}(40,:)'" : Constant  Value=[-0.34868091134588075075129154356545768678188323974609375;0.71163976165356579439702500167186371982097625732421875;2.25914385259164962604927495704032480716705322265625;0.1577562521924193161826366349487216211855411529541015625;-1.915798113589740836459895945154130458831787109375;1.38767243601959489041064443881623446941375732421875;-0.457821625679664945263169784084311686456203460693359375;-1.08565360321842252488977464963681995868682861328125;-0.682343662616461177350402067531831562519073486328125;-0.212814032725580914995333614569972269237041473388671875]
      mask Display: e = 0.06;c1 = [120 150 230]/255;c2 = ([120 150 230]+0)/383;c3 = ([120 150 230]+128)/383;patch([0 1 1 0],[0 0 1 1],c1);patch([0 1 1 1-e 1-e 0+e],[0 0 1 1-e 0+e 0+e],c2);patch([0 0 1 1-e 0+e 0+e],[0 1 1 1-e 1-e 0+e],c3);plot([0 1 1 0 0],[0 0 1 1 0]);disp('weights');
  "IW{2,1}(41,:)'" : Constant  Value=[-0.384693786478920163318662162055261433124542236328125;0.670405982836017155790386823355220258235931396484375;2.233547800532729610267779207788407802581787109375;0.29885623813081096944443970642169006168842315673828125;-1.1614848768459038463873866930953226983547210693359375;1.328849739927486783841459327959455549716949462890625;-0.57382634252319297818445420489297248423099517822265625;-0.50487318014105142527370162497390992939472198486328125;-1.2223651496305525387953139215824194252490997314453125;0.63080717880939707331577892546192742884159088134765625]
      mask Display: e = 0.06;c1 = [120 150 230]/255;c2 = ([120 150 230]+0)/383;c3 = ([120 150 230]+128)/383;patch([0 1 1 0],[0 0 1 1],c1);patch([0 1 1 1-e 1-e 0+e],[0 0 1 1-e 0+e 0+e],c2);patch([0 0 1 1-e 0+e 0+e],[0 1 1 1-e 1-e 0+e],c3);plot([0 1 1 0 0],[0 0 1 1 0]);disp('weights');
  "IW{2,1}(42,:)'" : Constant  Value=[-0.68954337845844893006841402893769554793834686279296875;0.76156028935077468844383474788628518581390380859375;2.733377962340927780360289034433662891387939453125;-0.3307189584512639779489973079762421548366546630859375;-1.767964860054358045005074018263258039951324462890625;1.7925680718506515898269526587682776153087615966796875;-0.05147072696549311043856533842699718661606311798095703125;-0.206982244610009080698631578343338333070278167724609375;0.11909077605025293611351600020498153753578662872314453125;1.152960876683140067910926518379710614681243896484375]
      mask Display: e = 0.06;c1 = [120 150 230]/255;c2 = ([120 150 230]+0)/383;c3 = ([120 150 230]+128)/383;patch([0 1 1 0],[0 0 1 1],c1);patch([0 1 1 1-e 1-e 0+e],[0 0 1 1-e 0+e 0+e],c2);patch([0 0 1 1-e 0+e 0+e],[0 1 1 1-e 1-e 0+e],c3);plot([0 1 1 0 0],[0 0 1 1 0]);disp('weights');
  "IW{2,1}(43,:)'" : Constant  Value=[-0.5929121540110366961329191326512955129146575927734375;0.70738919924875631739524806107510812580585479736328125;2.376005332543118075960819624015130102634429931640625;-0.76158579503022927337241299028391949832439422607421875;-2.10889938205355065292678773403167724609375;1.6506375691719892273567893425934016704559326171875;0.3913239221352433627743039323831908404827117919921875;0.10400934437467583559833173012521001510322093963623046875;-0.64661658623874285201083011997980065643787384033203125;0.69885919020168041360108190929167903959751129150390625]
      mask Display: e = 0.06;c1 = [120 150 230]/255;c2 = ([120 150 230]+0)/383;c3 = ([120 150 230]+128)/383;patch([0 1 1 0],[0 0 1 1],c1);patch([0 1 1 1-e 1-e 0+e],[0 0 1 1-e 0+e 0+e],c2);patch([0 0 1 1-e 0+e 0+e],[0 1 1 1-e 1-e 0+e],c3);plot([0 1 1 0 0],[0 0 1 1 0]);disp('weights');
  "IW{2,1}(44,:)'" : Constant  Value=[-0.0211814254701263859903548336660605855286121368408203125;0.5988864812756748978728182919439859688282012939453125;1.6910868744764149251835760878748260438442230224609375;0.40914415135783899213350878198980353772640228271484375;-1.895921791759112462472103288746438920497894287109375;0.9007222790673903300984193265321664512157440185546875;-0.61261974959761233971988758639781735837459564208984375;-0.301489605795037307611750065916567109525203704833984375;-1.3838127391879766481253000165452249348163604736328125;0.47532435357247226903609771397896111011505126953125]
      mask Display: e = 0.06;c1 = [120 150 230]/255;c2 = ([120 150 230]+0)/383;c3 = ([120 150 230]+128)/383;patch([0 1 1 0],[0 0 1 1],c1);patch([0 1 1 1-e 1-e 0+e],[0 0 1 1-e 0+e 0+e],c2);patch([0 0 1 1-e 0+e 0+e],[0 1 1 1-e 1-e 0+e],c3);plot([0 1 1 0 0],[0 0 1 1 0]);disp('weights');
  "IW{2,1}(45,:)'" : Constant  Value=[-0.57394830886734815589278468905831687152385711669921875;0.7758353840895348962902744460734538733959197998046875;2.729870216737170895981989815481938421726226806640625;0.486636550182550975396367221037507988512516021728515625;-1.73848539994374018391454228549264371395111083984375;1.6575732242535277105588420454296283423900604248046875;-0.819449929931143739025856120861135423183441162109375;-0.79445874364760593611123340451740659773349761962890625;0.062040531257998583758439536950390902347862720489501953125;0.5443755628008635216730226602521724998950958251953125]
      mask Display: e = 0.06;c1 = [120 150 230]/255;c2 = ([120 150 230]+0)/383;c3 = ([120 150 230]+128)/383;patch([0 1 1 0],[0 0 1 1],c1);patch([0 1 1 1-e 1-e 0+e],[0 0 1 1-e 0+e 0+e],c2);patch([0 0 1 1-e 0+e 0+e],[0 1 1 1-e 1-e 0+e],c3);plot([0 1 1 0 0],[0 0 1 1 0]);disp('weights');
  "IW{2,1}(46,:)'" : Constant  Value=[-0.41218791808006749466386509084259159862995147705078125;0.68294697094525858016567099184612743556499481201171875;2.1812169635464524475310099660418927669525146484375;-0.3122138439025423650718948920257389545440673828125;-2.3919144846367839107870167936198413372039794921875;1.4249365798424140638900325939175672829151153564453125;-0.005641744161312560283672024041834447416476905345916748046875;0.17410184172223341914076399916666559875011444091796875;-0.673316563070028184512239022296853363513946533203125;0.65772099647677573219795021941536106169223785400390625]
      mask Display: e = 0.06;c1 = [120 150 230]/255;c2 = ([120 150 230]+0)/383;c3 = ([120 150 230]+128)/383;patch([0 1 1 0],[0 0 1 1],c1);patch([0 1 1 1-e 1-e 0+e],[0 0 1 1-e 0+e 0+e],c2);patch([0 0 1 1-e 0+e 0+e],[0 1 1 1-e 1-e 0+e],c3);plot([0 1 1 0 0],[0 0 1 1 0]);disp('weights');
  "IW{2,1}(47,:)'" : Constant  Value=[-0.6601283821964922804426123548182658851146697998046875;0.71682210829467063462061560130678117275238037109375;2.507777607825319332590652265935204923152923583984375;-0.4691640106248977648562004105770029127597808837890625;-0.84098642960201963614252917977864854037761688232421875;1.6957724169771568600850741859176196157932281494140625;0.10582480693325056753106849782852805219590663909912109375;-0.97280418442449756444290187573642469942569732666015625;-1.334943670733434561981312072020955383777618408203125;0.078976933807087090766430037547252140939235687255859375]
      mask Display: e = 0.06;c1 = [120 150 230]/255;c2 = ([120 150 230]+0)/383;c3 = ([120 150 230]+128)/383;patch([0 1 1 0],[0 0 1 1],c1);patch([0 1 1 1-e 1-e 0+e],[0 0 1 1-e 0+e 0+e],c2);patch([0 0 1 1-e 0+e 0+e],[0 1 1 1-e 1-e 0+e],c3);plot([0 1 1 0 0],[0 0 1 1 0]);disp('weights');
  "IW{2,1}(48,:)'" : Constant  Value=[-0.456419298439418030799430425759055651724338531494140625;0.72313861048824179533767164684832096099853515625;2.40986742146247134854775140411220490932464599609375;0.0214512669821436165185080113815274671651422977447509765625;-1.19680450750258149383853378822095692157745361328125;1.5060527348488850218899415267514996230602264404296875;-0.34414919860015469321723458051565103232860565185546875;-1.482143618281361430177867077873088419437408447265625;-0.82798638096933807606347954788361676037311553955078125;-0.1802135218681593376022220809318241663277149200439453125]
      mask Display: e = 0.06;c1 = [120 150 230]/255;c2 = ([120 150 230]+0)/383;c3 = ([120 150 230]+128)/383;patch([0 1 1 0],[0 0 1 1],c1);patch([0 1 1 1-e 1-e 0+e],[0 0 1 1-e 0+e 0+e],c2);patch([0 0 1 1-e 0+e 0+e],[0 1 1 1-e 1-e 0+e],c3);plot([0 1 1 0 0],[0 0 1 1 0]);disp('weights');
  "IW{2,1}(49,:)'" : Constant  Value=[-0.201777420421350106582991656978265382349491119384765625;0.62191621841690125638280051134643144905567169189453125;1.8119283917398167904622141577419824898242950439453125;-0.5227232263910142062712793631362728774547576904296875;-2.439458773395342117140671689412556588649749755859375;1.1650190345772750699637754223658703267574310302734375;0.23989752362414018538316895501338876783847808837890625;0.205855921277374231959100825406494550406932830810546875;-0.9529096895648516696297747330390848219394683837890625;0.73215887561226222768340221591643057763576507568359375]
      mask Display: e = 0.06;c1 = [120 150 230]/255;c2 = ([120 150 230]+0)/383;c3 = ([120 150 230]+128)/383;patch([0 1 1 0],[0 0 1 1],c1);patch([0 1 1 1-e 1-e 0+e],[0 0 1 1-e 0+e 0+e],c2);patch([0 0 1 1-e 0+e 0+e],[0 1 1 1-e 1-e 0+e],c3);plot([0 1 1 0 0],[0 0 1 1 0]);disp('weights');
  "IW{2,1}(5,:)'" : Constant  Value=[-0.361104428885895167855579757087980397045612335205078125;0.63294787419499787262111567542888224124908447265625;2.070132619536046991726152555202133953571319580078125;0.420864372235277894862548464516294188797473907470703125;-1.485100440670633847872750266105867922306060791015625;1.25189228417873099630241995328105986118316650390625;-0.6766670609109386447244105511344969272613525390625;0.262109587209254535355995585632626898586750030517578125;-1.23739336927696097490070314961485564708709716796875;1.2100048860681276163830943914945237338542938232421875]
      mask Display: e = 0.06;c1 = [120 150 230]/255;c2 = ([120 150 230]+0)/383;c3 = ([120 150 230]+128)/383;patch([0 1 1 0],[0 0 1 1],c1);patch([0 1 1 1-e 1-e 0+e],[0 0 1 1-e 0+e 0+e],c2);patch([0 0 1 1-e 0+e 0+e],[0 1 1 1-e 1-e 0+e],c3);plot([0 1 1 0 0],[0 0 1 1 0]);disp('weights');
  "IW{2,1}(50,:)'" : Constant  Value=[-0.1710439451457241577525536513348924927413463592529296875;0.6582236969091852518687346673686988651752471923828125;2.011306021194341209223921396187506616115570068359375;0.38087735787934651199293512036092579364776611328125;-2.826802661426973894975844814325682818889617919921875;1.132059008564136437513525379472412168979644775390625;-0.6287175867037755327970671714865602552890777587890625;0.559666047608690764292305175331421196460723876953125;-0.154249598879783234028906235835165716707706451416015625;1.31421098450051854200637535541318356990814208984375]
      mask Display: e = 0.06;c1 = [120 150 230]/255;c2 = ([120 150 230]+0)/383;c3 = ([120 150 230]+128)/383;patch([0 1 1 0],[0 0 1 1],c1);patch([0 1 1 1-e 1-e 0+e],[0 0 1 1-e 0+e 0+e],c2);patch([0 0 1 1-e 0+e 0+e],[0 1 1 1-e 1-e 0+e],c3);plot([0 1 1 0 0],[0 0 1 1 0]);disp('weights');
  "IW{2,1}(51,:)'" : Constant  Value=[-0.79655882956646217873952764421119354665279388427734375;0.78415898119855464987182358527206815779209136962890625;2.91708511729693942271524065290577709674835205078125;-0.0223287146166207713104956411598323029465973377227783203125;-1.2530913987062886061352173783234320580959320068359375;1.8915671695448548206286432105116546154022216796875;-0.3616281011241284648605187612702138721942901611328125;-0.494062157839597226871575230688904412090778350830078125;-0.156785330838478065285102047710097394883632659912109375;0.926573513474272747458826415822841227054595947265625]
      mask Display: e = 0.06;c1 = [120 150 230]/255;c2 = ([120 150 230]+0)/383;c3 = ([120 150 230]+128)/383;patch([0 1 1 0],[0 0 1 1],c1);patch([0 1 1 1-e 1-e 0+e],[0 0 1 1-e 0+e 0+e],c2);patch([0 0 1 1-e 0+e 0+e],[0 1 1 1-e 1-e 0+e],c3);plot([0 1 1 0 0],[0 0 1 1 0]);disp('weights');
  "IW{2,1}(52,:)'" : Constant  Value=[-0.77520483877998980215551227956893853843212127685546875;0.77360216709961016068319850091938860714435577392578125;2.84526158862346445488356039277277886867523193359375;-0.124298281629053153363173578327405266463756561279296875;-1.3712902310571788433435358456335961818695068359375;1.8635474347286684615454532831790857017040252685546875;-0.258231915472281470247395418482483364641666412353515625;-0.38754152309492628791787183217820711433887481689453125;-0.25448599483401668219784141911077313125133514404296875;0.8858499832048656319472001996473409235477447509765625]
      mask Display: e = 0.06;c1 = [120 150 230]/255;c2 = ([120 150 230]+0)/383;c3 = ([120 150 230]+128)/383;patch([0 1 1 0],[0 0 1 1],c1);patch([0 1 1 1-e 1-e 0+e],[0 0 1 1-e 0+e 0+e],c2);patch([0 0 1 1-e 0+e 0+e],[0 1 1 1-e 1-e 0+e],c3);plot([0 1 1 0 0],[0 0 1 1 0]);disp('weights');
  "IW{2,1}(53,:)'" : Constant  Value=[0.0872313524475420154491445146049954928457736968994140625;0.56633619266558621330176492847385816276073455810546875;1.414107446701411863188013740000315010547637939453125;-0.1457789793707587044924167685167049057781696319580078125;-2.705267158957080031456143842660821974277496337890625;0.80225127206989110817403343389742076396942138671875;-0.06419827144783020467233569661402725614607334136962890625;0.1655860304536689309173880246817134320735931396484375;-1.29058179071715084518245930667035281658172607421875;0.487504541049491979531893548482912592589855194091796875]
      mask Display: e = 0.06;c1 = [120 150 230]/255;c2 = ([120 150 230]+0)/383;c3 = ([120 150 230]+128)/383;patch([0 1 1 0],[0 0 1 1],c1);patch([0 1 1 1-e 1-e 0+e],[0 0 1 1-e 0+e 0+e],c2);patch([0 0 1 1-e 0+e 0+e],[0 1 1 1-e 1-e 0+e],c3);plot([0 1 1 0 0],[0 0 1 1 0]);disp('weights');
  "IW{2,1}(54,:)'" : Constant  Value=[-0.23613096403390942956690423670806922018527984619140625;0.65529897595194419590569623323972336947917938232421875;2.033890023016687198520457968697883188724517822265625;0.404811655234107059531112327022128738462924957275390625;-1.6213718144730806525188882005750201642513275146484375;1.17408979967273108258041247609071433544158935546875;-0.65365531983297431306567659703432582318782806396484375;-0.630716979836520419411272087018005549907684326171875;-1.25046629090068694978299390641041100025177001953125;0.2077651995722728794913081173945101909339427947998046875]
      mask Display: e = 0.06;c1 = [120 150 230]/255;c2 = ([120 150 230]+0)/383;c3 = ([120 150 230]+128)/383;patch([0 1 1 0],[0 0 1 1],c1);patch([0 1 1 1-e 1-e 0+e],[0 0 1 1-e 0+e 0+e],c2);patch([0 0 1 1-e 0+e 0+e],[0 1 1 1-e 1-e 0+e],c3);plot([0 1 1 0 0],[0 0 1 1 0]);disp('weights');
  "IW{2,1}(55,:)'" : Constant  Value=[-0.316924737761261232638076990042463876307010650634765625;0.650890399474258973810947281890548765659332275390625;2.08746194188076827913391753099858760833740234375;0.54572230443555913570463644646224565804004669189453125;-1.53688837112396381456846938817761838436126708984375;1.216897312058887958841069121262989938259124755859375;-0.790321720203369437740548164583742618560791015625;-0.1283894583373827169570091655259602703154087066650390625;-1.556140172558479140008103058789856731891632080078125;0.440025672733066863795414747073664329946041107177734375]
      mask Display: e = 0.06;c1 = [120 150 230]/255;c2 = ([120 150 230]+0)/383;c3 = ([120 150 230]+128)/383;patch([0 1 1 0],[0 0 1 1],c1);patch([0 1 1 1-e 1-e 0+e],[0 0 1 1-e 0+e 0+e],c2);patch([0 0 1 1-e 0+e 0+e],[0 1 1 1-e 1-e 0+e],c3);plot([0 1 1 0 0],[0 0 1 1 0]);disp('weights');
  "IW{2,1}(56,:)'" : Constant  Value=[-0.3224581638423036356044804051634855568408966064453125;0.64905700226529716712065010142396204173564910888671875;2.0281504320326906309901460190303623676300048828125;-0.187224973364923663599057590545271523296833038330078125;-2.330806222918633263674337285920046269893646240234375;1.2814075613287199129075588643900118768215179443359375;-0.09959056565167816177375215147549170069396495819091796875;0.460901852520601729157334602859918959438800811767578125;-0.8883044940006084022598997762543149292469024658203125;0.95140959649191436664494858632679097354412078857421875]
      mask Display: e = 0.06;c1 = [120 150 230]/255;c2 = ([120 150 230]+0)/383;c3 = ([120 150 230]+128)/383;patch([0 1 1 0],[0 0 1 1],c1);patch([0 1 1 1-e 1-e 0+e],[0 0 1 1-e 0+e 0+e],c2);patch([0 0 1 1-e 0+e 0+e],[0 1 1 1-e 1-e 0+e],c3);plot([0 1 1 0 0],[0 0 1 1 0]);disp('weights');
  "IW{2,1}(57,:)'" : Constant  Value=[-0.12417800658433429672466985493883839808404445648193359375;0.63489238841727779760759631244582124054431915283203125;1.7787429116124580108504460440599359571933746337890625;-0.85761530530165652752572214012616313993930816650390625;-2.58550401206075974869236233644187450408935546875;1.15768441501506202939708600752055644989013671875;0.5545365864136593270217190365656279027462005615234375;-0.475925661700792812514038132576388306915760040283203125;-0.417279774207084896975317178657860495150089263916015625;0.4648503542820561218462671604356728494167327880859375]
      mask Display: e = 0.06;c1 = [120 150 230]/255;c2 = ([120 150 230]+0)/383;c3 = ([120 150 230]+128)/383;patch([0 1 1 0],[0 0 1 1],c1);patch([0 1 1 1-e 1-e 0+e],[0 0 1 1-e 0+e 0+e],c2);patch([0 0 1 1-e 0+e 0+e],[0 1 1 1-e 1-e 0+e],c3);plot([0 1 1 0 0],[0 0 1 1 0]);disp('weights');
  "IW{2,1}(58,:)'" : Constant  Value=[-0.408512290828903446016084899383713491261005401611328125;0.6903910850273968780044242521398700773715972900390625;2.255254765159134588969891410670243203639984130859375;-0.48586808559882010971620047712349332869052886962890625;-1.559833509795557571209201341844163835048675537109375;1.4524417495671244626720408632536418735980987548828125;0.1534105816325185556170396239394904114305973052978515625;-0.7944160430912792225655039146658964455127716064453125;-0.56777458726763063712184020914719440042972564697265625;0.56028111966335802929251030946034006774425506591796875]
      mask Display: e = 0.06;c1 = [120 150 230]/255;c2 = ([120 150 230]+0)/383;c3 = ([120 150 230]+128)/383;patch([0 1 1 0],[0 0 1 1],c1);patch([0 1 1 1-e 1-e 0+e],[0 0 1 1-e 0+e 0+e],c2);patch([0 0 1 1-e 0+e 0+e],[0 1 1 1-e 1-e 0+e],c3);plot([0 1 1 0 0],[0 0 1 1 0]);disp('weights');
  "IW{2,1}(59,:)'" : Constant  Value=[-0.6107556792473560758338635423569940030574798583984375;0.739678721840742792181799813988618552684783935546875;2.630413756708998906930219163768924772739410400390625;0.001501633270674982041648082287110810284502804279327392578125;-1.3060315221559182230492979215341620147228240966796875;1.6611833076681581378153396144625730812549591064453125;-0.34701328429750921689134202097193337976932525634765625;-0.54992402298263665105793052134686149656772613525390625;-0.39338078528469877515050256988615728914737701416015625;0.86903111347703287936639071631361730396747589111328125]
      mask Display: e = 0.06;c1 = [120 150 230]/255;c2 = ([120 150 230]+0)/383;c3 = ([120 150 230]+128)/383;patch([0 1 1 0],[0 0 1 1],c1);patch([0 1 1 1-e 1-e 0+e],[0 0 1 1-e 0+e 0+e],c2);patch([0 0 1 1-e 0+e 0+e],[0 1 1 1-e 1-e 0+e],c3);plot([0 1 1 0 0],[0 0 1 1 0]);disp('weights');
  "IW{2,1}(6,:)'" : Constant  Value=[-0.399290464443047887765914083502138964831829071044921875;0.65342796898937727245737505654687993228435516357421875;1.9708394281876489007032660083496011793613433837890625;0.318146478406188315535274568901513703167438507080078125;-2.014055302595394447706667051534168422222137451171875;1.3654105285378974610210889295558445155620574951171875;-0.6067339697149598531922265465254895389080047607421875;-0.71793312832606959172920824130414985120296478271484375;-1.2475937670573047366673336000530980527400970458984375;-0.275998356406463807299900281577720306813716888427734375]
      mask Display: e = 0.06;c1 = [120 150 230]/255;c2 = ([120 150 230]+0)/383;c3 = ([120 150 230]+128)/383;patch([0 1 1 0],[0 0 1 1],c1);patch([0 1 1 1-e 1-e 0+e],[0 0 1 1-e 0+e 0+e],c2);patch([0 0 1 1-e 0+e 0+e],[0 1 1 1-e 1-e 0+e],c3);plot([0 1 1 0 0],[0 0 1 1 0]);disp('weights');
  "IW{2,1}(60,:)'" : Constant  Value=[-0.7802368169402580377891354146413505077362060546875;0.81317539253569803836541041164309717714786529541015625;3.05386339398602757455591927282512187957763671875;0.4082729267082585433712438316433690488338470458984375;-1.3209612402571033751286222468479536473751068115234375;1.8964690309730893869044621169450692832469940185546875;-0.7814595882597263898361461542663164436817169189453125;-0.69594645287528134058874229594948701560497283935546875;0.331095172526763958931184106404543854296207427978515625;1.014523100757556139939197237254120409488677978515625]
      mask Display: e = 0.06;c1 = [120 150 230]/255;c2 = ([120 150 230]+0)/383;c3 = ([120 150 230]+128)/383;patch([0 1 1 0],[0 0 1 1],c1);patch([0 1 1 1-e 1-e 0+e],[0 0 1 1-e 0+e 0+e],c2);patch([0 0 1 1-e 0+e 0+e],[0 1 1 1-e 1-e 0+e],c3);plot([0 1 1 0 0],[0 0 1 1 0]);disp('weights');
  "IW{2,1}(61,:)'" : Constant  Value=[-0.1015364283458365102230658294502063654363155364990234375;0.64654327469720074272885312893777154386043548583984375;1.9061398192869207779409634895273484289646148681640625;0.63225229181944531120507235755212604999542236328125;-2.692639734177727728337004009517841041088104248046875;1.0333812915510820484854548340081237256526947021484375;-0.8535132018201923020939148045727051794528961181640625;0.21431775783098150345296062369015999138355255126953125;-0.59500476007141001044686845489195547997951507568359375;0.7643347368371899985817208289518021047115325927734375]
      mask Display: e = 0.06;c1 = [120 150 230]/255;c2 = ([120 150 230]+0)/383;c3 = ([120 150 230]+128)/383;patch([0 1 1 0],[0 0 1 1],c1);patch([0 1 1 1-e 1-e 0+e],[0 0 1 1-e 0+e 0+e],c2);patch([0 0 1 1-e 0+e 0+e],[0 1 1 1-e 1-e 0+e],c3);plot([0 1 1 0 0],[0 0 1 1 0]);disp('weights');
  "IW{2,1}(62,:)'" : Constant  Value=[-0.54190216643147104402800096067949198186397552490234375;0.74052847944521171807963355604442767798900604248046875;2.582187960433251827652156862313859164714813232421875;0.343741103102079781361766208647168241441249847412109375;-2.21727821415168246943494523293338716030120849609375;1.57915357807547263035985452006570994853973388671875;-0.664540738250165130551749825826846063137054443359375;0.2812971573694358351502842197078280150890350341796875;0.049693814115189284541518333071508095599710941314697265625;1.2803144120687728335639121723943389952182769775390625]
      mask Display: e = 0.06;c1 = [120 150 230]/255;c2 = ([120 150 230]+0)/383;c3 = ([120 150 230]+128)/383;patch([0 1 1 0],[0 0 1 1],c1);patch([0 1 1 1-e 1-e 0+e],[0 0 1 1-e 0+e 0+e],c2);patch([0 0 1 1-e 0+e 0+e],[0 1 1 1-e 1-e 0+e],c3);plot([0 1 1 0 0],[0 0 1 1 0]);disp('weights');
  "IW{2,1}(63,:)'" : Constant  Value=[-0.7313859295748386113444894363055936992168426513671875;0.85003606718380397833101369542418979108333587646484375;3.0847544502068249272497268975712358951568603515625;-0.1996454161762930834544960134735447354614734649658203125;-1.2806132223600361630388988487538881599903106689453125;1.979092292530915120352119629387743771076202392578125;-0.223519904872052699307261036665295250713825225830078125;-2.202488900502516333546054738690145313739776611328125;0.943420786240260600408191749011166393756866455078125;0.1106358584805301192854898317818879149854183197021484375]
      mask Display: e = 0.06;c1 = [120 150 230]/255;c2 = ([120 150 230]+0)/383;c3 = ([120 150 230]+128)/383;patch([0 1 1 0],[0 0 1 1],c1);patch([0 1 1 1-e 1-e 0+e],[0 0 1 1-e 0+e 0+e],c2);patch([0 0 1 1-e 0+e 0+e],[0 1 1 1-e 1-e 0+e],c3);plot([0 1 1 0 0],[0 0 1 1 0]);disp('weights');
  "IW{2,1}(64,:)'" : Constant  Value=[-0.5054205145860752868003373805549927055835723876953125;0.71417733125977067576428680695244111120700836181640625;2.3546600400439334777047406532801687717437744140625;-0.50845168097627990722031654513557441532611846923828125;-1.7696770735830380516517834621481597423553466796875;1.573089692838506525873754071653820574283599853515625;0.156123703682952197357991508397390134632587432861328125;-0.77066965724304703488911627573543228209018707275390625;-0.67931873722565006001872234264737926423549652099609375;0.152540870272499018422962535623810254037380218505859375]
      mask Display: e = 0.06;c1 = [120 150 230]/255;c2 = ([120 150 230]+0)/383;c3 = ([120 150 230]+128)/383;patch([0 1 1 0],[0 0 1 1],c1);patch([0 1 1 1-e 1-e 0+e],[0 0 1 1-e 0+e 0+e],c2);patch([0 0 1 1-e 0+e 0+e],[0 1 1 1-e 1-e 0+e],c3);plot([0 1 1 0 0],[0 0 1 1 0]);disp('weights');
  "IW{2,1}(65,:)'" : Constant  Value=[-0.280031881294614148902866190837812609970569610595703125;0.69377712158026760835838331331615336239337921142578125;2.1463085801865435797708414611406624317169189453125;-0.449439516098717961600783610265352763235569000244140625;-2.3308725413293789330282379523850977420806884765625;1.35486678672138527446122679975815117359161376953125;0.127376892280258002809745221384218893945217132568359375;-0.7265176063411222795451749334461055696010589599609375;-0.01317630460921424308262661639901125454343855381011962890625;0.51274706969753369723008518121787346899509429931640625]
      mask Display: e = 0.06;c1 = [120 150 230]/255;c2 = ([120 150 230]+0)/383;c3 = ([120 150 230]+128)/383;patch([0 1 1 0],[0 0 1 1],c1);patch([0 1 1 1-e 1-e 0+e],[0 0 1 1-e 0+e 0+e],c2);patch([0 0 1 1-e 0+e 0+e],[0 1 1 1-e 1-e 0+e],c3);plot([0 1 1 0 0],[0 0 1 1 0]);disp('weights');
  "IW{2,1}(66,:)'" : Constant  Value=[-0.07019409621359511131100106240410241298377513885498046875;0.6220313962611359048793246984132565557956695556640625;1.78335373214395787044850294478237628936767578125;-0.05823052063479221274189256973841111175715923309326171875;-2.37452077889735857496589233051054179668426513671875;1.0232739941724986465487745590507984161376953125;-0.18845769512102794607244504732079803943634033203125;-0.11497684349869684294898064536027959547936916351318359375;-0.62313085715640503803314231845433823764324188232421875;0.84528546262399106847595930958050303161144256591796875]
      mask Display: e = 0.06;c1 = [120 150 230]/255;c2 = ([120 150 230]+0)/383;c3 = ([120 150 230]+128)/383;patch([0 1 1 0],[0 0 1 1],c1);patch([0 1 1 1-e 1-e 0+e],[0 0 1 1-e 0+e 0+e],c2);patch([0 0 1 1-e 0+e 0+e],[0 1 1 1-e 1-e 0+e],c3);plot([0 1 1 0 0],[0 0 1 1 0]);disp('weights');
  "IW{2,1}(67,:)'" : Constant  Value=[-0.62963967763990036363708213684731163084506988525390625;0.6974977132055755202344471399555914103984832763671875;2.46385867011834580608820033376105129718780517578125;-0.306573921232210333531753576608025468885898590087890625;-1.0274874700000768967811382026411592960357666015625;1.6229587615866145622334215659066103398799896240234375;-0.035967329401550084122529682417734875343739986419677734375;-0.2386282825159083686994421213967143557965755462646484375;-1.206549460078165214582668340881355106830596923828125;0.8100935125724912921896248008124530315399169921875]
      mask Display: e = 0.06;c1 = [120 150 230]/255;c2 = ([120 150 230]+0)/383;c3 = ([120 150 230]+128)/383;patch([0 1 1 0],[0 0 1 1],c1);patch([0 1 1 1-e 1-e 0+e],[0 0 1 1-e 0+e 0+e],c2);patch([0 0 1 1-e 0+e 0+e],[0 1 1 1-e 1-e 0+e],c3);plot([0 1 1 0 0],[0 0 1 1 0]);disp('weights');
  "IW{2,1}(68,:)'" : Constant  Value=[-0.284932810080655851692199576064012944698333740234375;0.66378095421814720111797214485704898834228515625;2.074999478056641866174913957365788519382476806640625;-0.22732373441035502725782180277747102081775665283203125;-2.43281971157467324928802554495632648468017578125;1.2839498270414679836903815157711505889892578125;-0.06719123758005933477743809589810553006827831268310546875;0.2217783189529467235967530314155737869441509246826171875;-0.33138895880670560245562228374183177947998046875;1.122277486627905940252958316705189645290374755859375]
      mask Display: e = 0.06;c1 = [120 150 230]/255;c2 = ([120 150 230]+0)/383;c3 = ([120 150 230]+128)/383;patch([0 1 1 0],[0 0 1 1],c1);patch([0 1 1 1-e 1-e 0+e],[0 0 1 1-e 0+e 0+e],c2);patch([0 0 1 1-e 0+e 0+e],[0 1 1 1-e 1-e 0+e],c3);plot([0 1 1 0 0],[0 0 1 1 0]);disp('weights');
  "IW{2,1}(69,:)'" : Constant  Value=[0.01385211371534888526169115863240222097374498844146728515625;0.619465348974950646976367352181114256381988525390625;1.704004002652293348063494704547338187694549560546875;0.17028837879227520790692551599931903183460235595703125;-2.0447999645908652155412710271775722503662109375;0.932139487867977845070299736107699573040008544921875;-0.39526430104407006549394054673030041158199310302734375;-0.93951028378846712652006090138456784188747406005859375;-0.98689446375578271375417216404457576572895050048828125;0.06220454574006384351747556138434447348117828369140625]
      mask Display: e = 0.06;c1 = [120 150 230]/255;c2 = ([120 150 230]+0)/383;c3 = ([120 150 230]+128)/383;patch([0 1 1 0],[0 0 1 1],c1);patch([0 1 1 1-e 1-e 0+e],[0 0 1 1-e 0+e 0+e],c2);patch([0 0 1 1-e 0+e 0+e],[0 1 1 1-e 1-e 0+e],c3);plot([0 1 1 0 0],[0 0 1 1 0]);disp('weights');
  "IW{2,1}(7,:)'" : Constant  Value=[-0.276700442811016966704329433923703618347644805908203125;0.6809882664322746137486319639720022678375244140625;2.227162799561631434386299588368274271488189697265625;0.01014526067216965643513759687266428954899311065673828125;-1.9549257907233250630696375083061866462230682373046875;1.2354837515605259223860912243253551423549652099609375;-0.277545927745709519740557880140841007232666015625;0.27650282940929848951583380767260678112506866455078125;-1.0067512224415808841371244852780364453792572021484375;0.8787308430758555832795764217735268175601959228515625]
      mask Display: e = 0.06;c1 = [120 150 230]/255;c2 = ([120 150 230]+0)/383;c3 = ([120 150 230]+128)/383;patch([0 1 1 0],[0 0 1 1],c1);patch([0 1 1 1-e 1-e 0+e],[0 0 1 1-e 0+e 0+e],c2);patch([0 0 1 1-e 0+e 0+e],[0 1 1 1-e 1-e 0+e],c3);plot([0 1 1 0 0],[0 0 1 1 0]);disp('weights');
  "IW{2,1}(70,:)'" : Constant  Value=[-0.2991403865439068443521364315529353916645050048828125;0.67234087069133774416940241280826739966869354248046875;2.00937246136564251486333887442015111446380615234375;-0.59146493629497298716302111643017269670963287353515625;-2.608811726607654701837191169033758342266082763671875;1.3400945344689054739006905947462655603885650634765625;0.272147668798055464289831206770031712949275970458984375;-0.315966385488408663118065078379004262387752532958984375;-0.64032293068934154067761710393824614584445953369140625;0.1431423776117629886872606448378064669668674468994140625]
      mask Display: e = 0.06;c1 = [120 150 230]/255;c2 = ([120 150 230]+0)/383;c3 = ([120 150 230]+128)/383;patch([0 1 1 0],[0 0 1 1],c1);patch([0 1 1 1-e 1-e 0+e],[0 0 1 1-e 0+e 0+e],c2);patch([0 0 1 1-e 0+e 0+e],[0 1 1 1-e 1-e 0+e],c3);plot([0 1 1 0 0],[0 0 1 1 0]);disp('weights');
  "IW{2,1}(71,:)'" : Constant  Value=[-0.2399291388015728221372313555548316799104213714599609375;0.63699290910733818993350041637313552200794219970703125;1.935444199788679764395737947779707610607147216796875;-0.320363185556961582722834691594471223652362823486328125;-1.662335780870591417368586917291395366191864013671875;1.205917609285120928319656741223298013210296630859375;0.038352402176459431115684850510660908184945583343505859375;-0.57356170643615433935025293976650573313236236572265625;-1.162376468580807564734413972473703324794769287109375;0.4039263887989912316101026590331457555294036865234375]
      mask Display: e = 0.06;c1 = [120 150 230]/255;c2 = ([120 150 230]+0)/383;c3 = ([120 150 230]+128)/383;patch([0 1 1 0],[0 0 1 1],c1);patch([0 1 1 1-e 1-e 0+e],[0 0 1 1-e 0+e 0+e],c2);patch([0 0 1 1-e 0+e 0+e],[0 1 1 1-e 1-e 0+e],c3);plot([0 1 1 0 0],[0 0 1 1 0]);disp('weights');
  "IW{2,1}(72,:)'" : Constant  Value=[-0.311596947669967538896429459782666526734828948974609375;0.610707441228039105141078835004009306430816650390625;1.87034116106754222386143737821839749813079833984375;-0.61668700467854697944147801536018960177898406982421875;-1.6097341288991444674394415415008552372455596923828125;1.238074485576662997488028850057162344455718994140625;0.325785556900613004760458579767146147787570953369140625;0.04728371036911539759817202366320998407900333404541015625;-1.6496912833488182048569115067948587238788604736328125;0.65438448431920814840623279451392590999603271484375]
      mask Display: e = 0.06;c1 = [120 150 230]/255;c2 = ([120 150 230]+0)/383;c3 = ([120 150 230]+128)/383;patch([0 1 1 0],[0 0 1 1],c1);patch([0 1 1 1-e 1-e 0+e],[0 0 1 1-e 0+e 0+e],c2);patch([0 0 1 1-e 0+e 0+e],[0 1 1 1-e 1-e 0+e],c3);plot([0 1 1 0 0],[0 0 1 1 0]);disp('weights');
  "IW{2,1}(73,:)'" : Constant  Value=[-0.7209500876330678931225293126772157847881317138671875;0.755763415033980923141143648535944521427154541015625;2.689325131170086091714210851932875812053680419921875;-0.816217120382922711741002785856835544109344482421875;-1.862369012929210310147709606098942458629608154296875;1.8475739936683945874307255508028902113437652587890625;0.406878177218028158623752688072272576391696929931640625;-0.171322123933113801275140986035694368183612823486328125;0.08332371247354437848731123494872008450329303741455078125;1.094089992287494705891504054307006299495697021484375]
      mask Display: e = 0.06;c1 = [120 150 230]/255;c2 = ([120 150 230]+0)/383;c3 = ([120 150 230]+128)/383;patch([0 1 1 0],[0 0 1 1],c1);patch([0 1 1 1-e 1-e 0+e],[0 0 1 1-e 0+e 0+e],c2);patch([0 0 1 1-e 0+e 0+e],[0 1 1 1-e 1-e 0+e],c3);plot([0 1 1 0 0],[0 0 1 1 0]);disp('weights');
  "IW{2,1}(74,:)'" : Constant  Value=[0.2976311724445144246686822953051887452602386474609375;0.531793632804808513725447483011521399021148681640625;1.0576753577133086725581279097241349518299102783203125;-0.7131894776826002146918881408055312931537628173828125;-3.217474879370787466115189090487547218799591064453125;0.62123171786160591434367006513639353215694427490234375;0.5049550880845778966232728635077364742755889892578125;-0.2489369362560658049954298576267319731414318084716796875;-1.2108032797405898772780119543313048779964447021484375;-0.0212933392709513218121752942124658147804439067840576171875]
      mask Display: e = 0.06;c1 = [120 150 230]/255;c2 = ([120 150 230]+0)/383;c3 = ([120 150 230]+128)/383;patch([0 1 1 0],[0 0 1 1],c1);patch([0 1 1 1-e 1-e 0+e],[0 0 1 1-e 0+e 0+e],c2);patch([0 0 1 1-e 0+e 0+e],[0 1 1 1-e 1-e 0+e],c3);plot([0 1 1 0 0],[0 0 1 1 0]);disp('weights');
  "IW{2,1}(75,:)'" : Constant  Value=[-0.27720756424010872809304828479071147739887237548828125;0.650481283311116431633536194567568600177764892578125;2.078324912596803297759606721228919923305511474609375;0.0063501059279374542920759694197840872220695018768310546875;-2.11765003497412518385090152150951325893402099609375;1.2337927561101287299294426702545024454593658447265625;-0.28058358787081461027668183305650018155574798583984375;0.3996613459875881790850371544365771114826202392578125;-0.47993063630082632986528778928914107382297515869140625;1.4758181294987442466748461811221204698085784912109375]
      mask Display: e = 0.06;c1 = [120 150 230]/255;c2 = ([120 150 230]+0)/383;c3 = ([120 150 230]+128)/383;patch([0 1 1 0],[0 0 1 1],c1);patch([0 1 1 1-e 1-e 0+e],[0 0 1 1-e 0+e 0+e],c2);patch([0 0 1 1-e 0+e 0+e],[0 1 1 1-e 1-e 0+e],c3);plot([0 1 1 0 0],[0 0 1 1 0]);disp('weights');
  "IW{2,1}(76,:)'" : Constant  Value=[-0.290489399619584698353236262846621684730052947998046875;0.65333704263307301740582033744431100785732269287109375;2.043692431390223163134578499011695384979248046875;-0.31429130535998905937589142922661267220973968505859375;-1.92233804854541379114607480005361139774322509765625;1.276051502537221882249696136568672955036163330078125;0.0198778411494612526622116632779579958878457546234130859375;-0.2038734712536803550531061546280398033559322357177734375;-0.746864783769186857398381107486784458160400390625;0.82361151639543772606799620916717685759067535400390625]
      mask Display: e = 0.06;c1 = [120 150 230]/255;c2 = ([120 150 230]+0)/383;c3 = ([120 150 230]+128)/383;patch([0 1 1 0],[0 0 1 1],c1);patch([0 1 1 1-e 1-e 0+e],[0 0 1 1-e 0+e 0+e],c2);patch([0 0 1 1-e 0+e 0+e],[0 1 1 1-e 1-e 0+e],c3);plot([0 1 1 0 0],[0 0 1 1 0]);disp('weights');
  "IW{2,1}(77,:)'" : Constant  Value=[-0.2403708345905925247709689074326888658106327056884765625;0.660595307100141582168362219817936420440673828125;2.09476738403838513846721980371512472629547119140625;0.339759083666326233696963754482567310333251953125;-1.4451723417483324229948493666597642004489898681640625;1.1942566052560106282243168607237748801708221435546875;-0.5963701359873738727657155322958715260028839111328125;-0.72701947997721660943426513767917640507221221923828125;-0.9358749847514713504637029473087750375270843505859375;0.54825352609675037651726370313554070889949798583984375]
      mask Display: e = 0.06;c1 = [120 150 230]/255;c2 = ([120 150 230]+0)/383;c3 = ([120 150 230]+128)/383;patch([0 1 1 0],[0 0 1 1],c1);patch([0 1 1 1-e 1-e 0+e],[0 0 1 1-e 0+e 0+e],c2);patch([0 0 1 1-e 0+e 0+e],[0 1 1 1-e 1-e 0+e],c3);plot([0 1 1 0 0],[0 0 1 1 0]);disp('weights');
  "IW{2,1}(78,:)'" : Constant  Value=[-0.285678120484556818947652345741516910493373870849609375;0.69367739688160157118801407705177552998065948486328125;2.209309789020462932995769733679480850696563720703125;0.5268072537339831828973046867758966982364654541015625;-2.14083425219214262824607430957257747650146484375;1.27445060203948656862849020399153232574462890625;-0.79245830372026004884133953964919783174991607666015625;-0.389533992546670315704204767826013267040252685546875;-0.5163631576529468247827026061713695526123046875;0.487064717297016780417351355936261825263500213623046875]
      mask Display: e = 0.06;c1 = [120 150 230]/255;c2 = ([120 150 230]+0)/383;c3 = ([120 150 230]+128)/383;patch([0 1 1 0],[0 0 1 1],c1);patch([0 1 1 1-e 1-e 0+e],[0 0 1 1-e 0+e 0+e],c2);patch([0 0 1 1-e 0+e 0+e],[0 1 1 1-e 1-e 0+e],c3);plot([0 1 1 0 0],[0 0 1 1 0]);disp('weights');
  "IW{2,1}(79,:)'" : Constant  Value=[0.338718635692556058192081991364830173552036285400390625;0.5448804037594265903265977613045834004878997802734375;1.160875924932642799802806621300987899303436279296875;-0.05508332293890776110156792810812476091086864471435546875;-3.3975560483573872261331416666507720947265625;0.5582911464461981498885734254145063459873199462890625;-0.11978456558838974921332720668942783959209918975830078125;0.1365966963327045480269816835061646997928619384765625;-0.7037847180006260305873411198263056576251983642578125;0.60427070429837892451274683480733074247837066650390625]
      mask Display: e = 0.06;c1 = [120 150 230]/255;c2 = ([120 150 230]+0)/383;c3 = ([120 150 230]+128)/383;patch([0 1 1 0],[0 0 1 1],c1);patch([0 1 1 1-e 1-e 0+e],[0 0 1 1-e 0+e 0+e],c2);patch([0 0 1 1-e 0+e 0+e],[0 1 1 1-e 1-e 0+e],c3);plot([0 1 1 0 0],[0 0 1 1 0]);disp('weights');
  "IW{2,1}(8,:)'" : Constant  Value=[-0.34882636042262615827524996348074637353420257568359375;0.6768046679267112342159862237167544662952423095703125;2.20397362534585194993042023270390927791595458984375;-0.025949597515031765093684867906631552614271640777587890625;-1.6957019800647241680735533009283244609832763671875;1.3705353811117915174833115088404156267642974853515625;-0.280841745611812687588582093667355366051197052001953125;-0.590940669586502931309723862796090543270111083984375;-0.01480401355286268573474561804914628737606108188629150390625;1.2229875034588391091716630398877896368503570556640625]
      mask Display: e = 0.06;c1 = [120 150 230]/255;c2 = ([120 150 230]+0)/383;c3 = ([120 150 230]+128)/383;patch([0 1 1 0],[0 0 1 1],c1);patch([0 1 1 1-e 1-e 0+e],[0 0 1 1-e 0+e 0+e],c2);patch([0 0 1 1-e 0+e 0+e],[0 1 1 1-e 1-e 0+e],c3);plot([0 1 1 0 0],[0 0 1 1 0]);disp('weights');
  "IW{2,1}(80,:)'" : Constant  Value=[-0.26137160426438510452129548866651020944118499755859375;0.65746672419112062168977672627079300582408905029296875;1.9641263793430783213267432074644602835178375244140625;-0.569244475147243189638857074896804988384246826171875;-2.201934173112239268021994575974531471729278564453125;1.2815722429934688353370120239560492336750030517578125;0.261256173633013677459757673204876482486724853515625;-0.55172607030371001446411582946893759071826934814453125;-0.801045785389949305255186118301935493946075439453125;0.205731910752760704941266567402635701000690460205078125]
      mask Display: e = 0.06;c1 = [120 150 230]/255;c2 = ([120 150 230]+0)/383;c3 = ([120 150 230]+128)/383;patch([0 1 1 0],[0 0 1 1],c1);patch([0 1 1 1-e 1-e 0+e],[0 0 1 1-e 0+e 0+e],c2);patch([0 0 1 1-e 0+e 0+e],[0 1 1 1-e 1-e 0+e],c3);plot([0 1 1 0 0],[0 0 1 1 0]);disp('weights');
  "IW{2,1}(81,:)'" : Constant  Value=[0.1500151726946044872246233126134029589593410491943359375;0.5878068945228223096677311332314275205135345458984375;1.495745505782296813634957288741134107112884521484375;0.534655419397717768248412539833225309848785400390625;-2.6470507944549961365510171162895858287811279296875;0.734779824315872520656967026297934353351593017578125;-0.71163960895488875824099750388995744287967681884765625;-0.219913527898424054907167146666324697434902191162109375;-1.0775358071536829118741707134176976978778839111328125;0.299111607184940175852005950218881480395793914794921875]
      mask Display: e = 0.06;c1 = [120 150 230]/255;c2 = ([120 150 230]+0)/383;c3 = ([120 150 230]+128)/383;patch([0 1 1 0],[0 0 1 1],c1);patch([0 1 1 1-e 1-e 0+e],[0 0 1 1-e 0+e 0+e],c2);patch([0 0 1 1-e 0+e 0+e],[0 1 1 1-e 1-e 0+e],c3);plot([0 1 1 0 0],[0 0 1 1 0]);disp('weights');
  "IW{2,1}(82,:)'" : Constant  Value=[-0.1265424492260665001452935030101798474788665771484375;0.58506864677448711109519763340358622372150421142578125;1.6330608443247973671219597235904075205326080322265625;0.0925893820267945921731467251447611488401889801025390625;-2.574652951732170347298733759089373052120208740234375;0.98300016451911365056304248355445452034473419189453125;-0.31421525244029469003947951932786963880062103271484375;0.83892382385926900223438451575930230319499969482421875;-1.731302077753896551115531110554002225399017333984375;0.63511018365878946223546108740265481173992156982421875]
      mask Display: e = 0.06;c1 = [120 150 230]/255;c2 = ([120 150 230]+0)/383;c3 = ([120 150 230]+128)/383;patch([0 1 1 0],[0 0 1 1],c1);patch([0 1 1 1-e 1-e 0+e],[0 0 1 1-e 0+e 0+e],c2);patch([0 0 1 1-e 0+e 0+e],[0 1 1 1-e 1-e 0+e],c3);plot([0 1 1 0 0],[0 0 1 1 0]);disp('weights');
  "IW{2,1}(83,:)'" : Constant  Value=[-0.430848918534638636312905646263970993459224700927734375;0.66534392666924657699922818210325203835964202880859375;2.16167373004275731318557518534362316131591796875;-0.319675704702803431533908451456227339804172515869140625;-1.269102624015985281147322893957607448101043701171875;1.4074283350143357296246904297731816768646240234375;0.0090119354554479558228052837876020930707454681396484375;-0.64746638783863030841558838801574893295764923095703125;-1.4717509327023827747638051732792519032955169677734375;0.1864505360238669362527019757180823944509029388427734375]
      mask Display: e = 0.06;c1 = [120 150 230]/255;c2 = ([120 150 230]+0)/383;c3 = ([120 150 230]+128)/383;patch([0 1 1 0],[0 0 1 1],c1);patch([0 1 1 1-e 1-e 0+e],[0 0 1 1-e 0+e 0+e],c2);patch([0 0 1 1-e 0+e 0+e],[0 1 1 1-e 1-e 0+e],c3);plot([0 1 1 0 0],[0 0 1 1 0]);disp('weights');
  "IW{2,1}(84,:)'" : Constant  Value=[-0.139025124727237325839013237782637588679790496826171875;0.68814345025193690563725112951942719519138336181640625;2.073281784946398698110670011374168097972869873046875;0.182807108080324909327174509598989970982074737548828125;-2.753653768053162753659535155748017132282257080078125;1.1801134873803322822283234927454032003879547119140625;-0.455021035647405647228680436455761082470417022705078125;-0.434539327895173410620799359094235114753246307373046875;0.30073491383447981117882363832904957234859466552734375;0.77744119352690599367150525722536258399486541748046875]
      mask Display: e = 0.06;c1 = [120 150 230]/255;c2 = ([120 150 230]+0)/383;c3 = ([120 150 230]+128)/383;patch([0 1 1 0],[0 0 1 1],c1);patch([0 1 1 1-e 1-e 0+e],[0 0 1 1-e 0+e 0+e],c2);patch([0 0 1 1-e 0+e 0+e],[0 1 1 1-e 1-e 0+e],c3);plot([0 1 1 0 0],[0 0 1 1 0]);disp('weights');
  "IW{2,1}(85,:)'" : Constant  Value=[-0.32557430977520718240469932425185106694698333740234375;0.6346546733568256826174547313712537288665771484375;1.99254675072523301793125938274897634983062744140625;-0.406934636369170099623460146176512353122234344482421875;-1.7628665224858384164008384686894714832305908203125;1.276208353662455774468753588735125958919525146484375;0.114345532425314255764448034824454225599765777587890625;0.06037876974145763020462851500269607640802860260009765625;-1.19281974349131747459296093438751995563507080078125;0.852919266095857775411559487110935151576995849609375]
      mask Display: e = 0.06;c1 = [120 150 230]/255;c2 = ([120 150 230]+0)/383;c3 = ([120 150 230]+128)/383;patch([0 1 1 0],[0 0 1 1],c1);patch([0 1 1 1-e 1-e 0+e],[0 0 1 1-e 0+e 0+e],c2);patch([0 0 1 1-e 0+e 0+e],[0 1 1 1-e 1-e 0+e],c3);plot([0 1 1 0 0],[0 0 1 1 0]);disp('weights');
  "IW{2,1}(86,:)'" : Constant  Value=[-0.04992622597242790671856482731527648866176605224609375;0.5263335589573963080312068996136076748371124267578125;1.34120486099081848152536622365005314350128173828125;-0.8690742485525617677666332383523695170879364013671875;-2.308217729927935391032178813475184142589569091796875;0.89716954257680769924121477743028663098812103271484375;0.6272906860750868673903823946602642536163330078125;0.8350893809115029764456039629294537007808685302734375;-2.019174002417118085617175893275998532772064208984375;0.89807662986151559625369600325939245522022247314453125]
      mask Display: e = 0.06;c1 = [120 150 230]/255;c2 = ([120 150 230]+0)/383;c3 = ([120 150 230]+128)/383;patch([0 1 1 0],[0 0 1 1],c1);patch([0 1 1 1-e 1-e 0+e],[0 0 1 1-e 0+e 0+e],c2);patch([0 0 1 1-e 0+e 0+e],[0 1 1 1-e 1-e 0+e],c3);plot([0 1 1 0 0],[0 0 1 1 0]);disp('weights');
  "IW{2,1}(87,:)'" : Constant  Value=[-0.82365722529714469057893211356713436543941497802734375;0.7794595941683464257465629998478107154369354248046875;2.85753325328157803397743919049389660358428955078125;-0.68944554083995635007653390857740305364131927490234375;-1.73509711264531940599908921285532414913177490234375;1.96114269916867112186764643411152064800262451171875;0.267424946120029705109999440537649206817150115966796875;-0.1440431754100112982097670055736671201884746551513671875;0.11687627132871460100549398930525057949125766754150390625;1.1161455302173306503021876778802834451198577880859375]
      mask Display: e = 0.06;c1 = [120 150 230]/255;c2 = ([120 150 230]+0)/383;c3 = ([120 150 230]+128)/383;patch([0 1 1 0],[0 0 1 1],c1);patch([0 1 1 1-e 1-e 0+e],[0 0 1 1-e 0+e 0+e],c2);patch([0 0 1 1-e 0+e 0+e],[0 1 1 1-e 1-e 0+e],c3);plot([0 1 1 0 0],[0 0 1 1 0]);disp('weights');
  "IW{2,1}(88,:)'" : Constant  Value=[0.01133323586675085391239914400784982717595994472503662109375;0.6232198410171314595373814881895668804645538330078125;1.673922251294841512248012804775498807430267333984375;-0.08566552143115709061493845410950598306953907012939453125;-2.486747620470645347978688732837326824665069580078125;0.9627964844777856523450054737622849643230438232421875;-0.15592903182438566656031753154820762574672698974609375;-0.74887134897027618496423428950947709381580352783203125;-0.7778933435063521972807620841194875538349151611328125;0.040774210652151317291203014292477746494114398956298828125]
      mask Display: e = 0.06;c1 = [120 150 230]/255;c2 = ([120 150 230]+0)/383;c3 = ([120 150 230]+128)/383;patch([0 1 1 0],[0 0 1 1],c1);patch([0 1 1 1-e 1-e 0+e],[0 0 1 1-e 0+e 0+e],c2);patch([0 0 1 1-e 0+e 0+e],[0 1 1 1-e 1-e 0+e],c3);plot([0 1 1 0 0],[0 0 1 1 0]);disp('weights');
  "IW{2,1}(89,:)'" : Constant  Value=[-0.397695794850412676080253504551365040242671966552734375;0.7192089133690038327273441609577275812625885009765625;2.38797062596876497053699495154432952404022216796875;0.6989853240521337607304985795053653419017791748046875;-1.145200212929535776851253103814087808132171630859375;1.39411380408798546426396569586358964443206787109375;-0.97573217415818092046464471422950737178325653076171875;-1.4499391558874830110426046303473412990570068359375;-1.1091085974754137932762887430726550519466400146484375;-0.348761644239788115573475124620017595589160919189453125]
      mask Display: e = 0.06;c1 = [120 150 230]/255;c2 = ([120 150 230]+0)/383;c3 = ([120 150 230]+128)/383;patch([0 1 1 0],[0 0 1 1],c1);patch([0 1 1 1-e 1-e 0+e],[0 0 1 1-e 0+e 0+e],c2);patch([0 0 1 1-e 0+e 0+e],[0 1 1 1-e 1-e 0+e],c3);plot([0 1 1 0 0],[0 0 1 1 0]);disp('weights');
  "IW{2,1}(9,:)'" : Constant  Value=[-0.03451339624112924331367224795030779205262660980224609375;0.575441627105979680578684565261937677860260009765625;1.55409236701997155449817000771872699260711669921875;-0.67260011948454689889587143625249154865741729736328125;-2.386918166573584354495096704340539872646331787109375;0.96729451918264131027314078892231918871402740478515625;0.414593815730289083631987523403950035572052001953125;0.1967897729899218128846172248813672922551631927490234375;-0.87467971892427243130185843256185762584209442138671875;1.1139111226895661577174223566544242203235626220703125]
      mask Display: e = 0.06;c1 = [120 150 230]/255;c2 = ([120 150 230]+0)/383;c3 = ([120 150 230]+128)/383;patch([0 1 1 0],[0 0 1 1],c1);patch([0 1 1 1-e 1-e 0+e],[0 0 1 1-e 0+e 0+e],c2);patch([0 0 1 1-e 0+e 0+e],[0 1 1 1-e 1-e 0+e],c3);plot([0 1 1 0 0],[0 0 1 1 0]);disp('weights');
  "IW{2,1}(90,:)'" : Constant  Value=[-0.52935195525594724852425088101881556212902069091796875;0.74514238197956228493268326928955502808094024658203125;2.570947260701955894290904325316660106182098388671875;0.039413737408720901644887391057636705227196216583251953125;-1.569698109141244746211896199383772909641265869140625;1.60396703394869977188363918685354292392730712890625;-0.37895884435160731573688508433406241238117218017578125;-0.86233022215031118751227268148795701563358306884765625;-0.1745734792227644771589467609373969025909900665283203125;0.5651449250821618530693513093865476548671722412109375]
      mask Display: e = 0.06;c1 = [120 150 230]/255;c2 = ([120 150 230]+0)/383;c3 = ([120 150 230]+128)/383;patch([0 1 1 0],[0 0 1 1],c1);patch([0 1 1 1-e 1-e 0+e],[0 0 1 1-e 0+e 0+e],c2);patch([0 0 1 1-e 0+e 0+e],[0 1 1 1-e 1-e 0+e],c3);plot([0 1 1 0 0],[0 0 1 1 0]);disp('weights');
  "IW{2,1}(91,:)'" : Constant  Value=[-0.64572068774630952958659690921194851398468017578125;0.68116210206111882374813148999237455427646636962890625;2.3886716464062747178331846953369677066802978515625;-0.817123628691332815066061812103725969791412353515625;-1.168440987061918345801814211881719529628753662109375;1.6492722320525736723340060052578337490558624267578125;0.452038713333215991241331721539609134197235107421875;0.06269932915319538502263441159811918623745441436767578125;-1.173542886420702924255010657361708581447601318359375;1.0742942495251075474271829079953022301197052001953125]
      mask Display: e = 0.06;c1 = [120 150 230]/255;c2 = ([120 150 230]+0)/383;c3 = ([120 150 230]+128)/383;patch([0 1 1 0],[0 0 1 1],c1);patch([0 1 1 1-e 1-e 0+e],[0 0 1 1-e 0+e 0+e],c2);patch([0 0 1 1-e 0+e 0+e],[0 1 1 1-e 1-e 0+e],c3);plot([0 1 1 0 0],[0 0 1 1 0]);disp('weights');
  "IW{2,1}(92,:)'" : Constant  Value=[-0.284024662979844022547837312231422401964664459228515625;0.6417780217508333162612643718603067100048065185546875;1.9168624157083129500023233049432747066020965576171875;-0.93615246544382946236595444133854471147060394287109375;-2.195218974490393382126285359845496714115142822265625;1.3020522052445269167719743563793599605560302734375;0.61293907419799709135332932419260032474994659423828125;-0.26534930435083692312758785192272625863552093505859375;-0.82811075833256264644433031207881867885589599609375;0.5189648536585853566549531024065800011157989501953125]
      mask Display: e = 0.06;c1 = [120 150 230]/255;c2 = ([120 150 230]+0)/383;c3 = ([120 150 230]+128)/383;patch([0 1 1 0],[0 0 1 1],c1);patch([0 1 1 1-e 1-e 0+e],[0 0 1 1-e 0+e 0+e],c2);patch([0 0 1 1-e 0+e 0+e],[0 1 1 1-e 1-e 0+e],c3);plot([0 1 1 0 0],[0 0 1 1 0]);disp('weights');
  "IW{2,1}(93,:)'" : Constant  Value=[-0.2354513356598309237188715314914588816463947296142578125;0.6557285425894698871474020052119158208370208740234375;2.08284222736943291920397314243018627166748046875;0.489609150445258156647554415030754171311855316162109375;-2.357875514824311569128667542827315628528594970703125;1.1688763334128611237616723883547820150852203369140625;-0.73513494966071324387968388691660948097705841064453125;0.57440085632705206730719282859354279935359954833984375;-0.450221203588835272579871116249705664813518524169921875;1.4384260970477991126159622581326402723789215087890625]
      mask Display: e = 0.06;c1 = [120 150 230]/255;c2 = ([120 150 230]+0)/383;c3 = ([120 150 230]+128)/383;patch([0 1 1 0],[0 0 1 1],c1);patch([0 1 1 1-e 1-e 0+e],[0 0 1 1-e 0+e 0+e],c2);patch([0 0 1 1-e 0+e 0+e],[0 1 1 1-e 1-e 0+e],c3);plot([0 1 1 0 0],[0 0 1 1 0]);disp('weights');
  "IW{2,1}(94,:)'" : Constant  Value=[-0.40654158390018368951501770425238646566867828369140625;0.65468392938205621778280374201131053268909454345703125;2.02860338354710023622828884981572628021240234375;-0.9863931009287083551129171610227786004543304443359375;-1.65690798908319347759743322967551648616790771484375;1.4253136106163599716722956145531497895717620849609375;0.645015050341998463778736550011672079563140869140625;-0.66719369310090426150594566934159956872463226318359375;-1.3648211872714901549130672719911672174930572509765625;0.003293365924245232785605441705456541967578232288360595703125]
      mask Display: e = 0.06;c1 = [120 150 230]/255;c2 = ([120 150 230]+0)/383;c3 = ([120 150 230]+128)/383;patch([0 1 1 0],[0 0 1 1],c1);patch([0 1 1 1-e 1-e 0+e],[0 0 1 1-e 0+e 0+e],c2);patch([0 0 1 1-e 0+e 0+e],[0 1 1 1-e 1-e 0+e],c3);plot([0 1 1 0 0],[0 0 1 1 0]);disp('weights');
  "IW{2,1}(95,:)'" : Constant  Value=[-0.337528224679392641061070889918482862412929534912109375;0.62333359894304563031397492522955872118473052978515625;1.8962466368408847916526838162099011242389678955078125;-0.69005906021558016671946234055212698876857757568359375;-2.088463318477530084038562563364394009113311767578125;1.287550646771443485505415083025582134723663330078125;0.38690593249583182799966607490205205976963043212890625;0.326295361317667842460110705360420979559421539306640625;-1.4315910226424513052023712589289061725139617919921875;0.639351250924150793508715651114471256732940673828125]
      mask Display: e = 0.06;c1 = [120 150 230]/255;c2 = ([120 150 230]+0)/383;c3 = ([120 150 230]+128)/383;patch([0 1 1 0],[0 0 1 1],c1);patch([0 1 1 1-e 1-e 0+e],[0 0 1 1-e 0+e 0+e],c2);patch([0 0 1 1-e 0+e 0+e],[0 1 1 1-e 1-e 0+e],c3);plot([0 1 1 0 0],[0 0 1 1 0]);disp('weights');
  "IW{2,1}(96,:)'" : Constant  Value=[-0.478441518821944689054959098939434625208377838134765625;0.77872676515633632021717858151532709598541259765625;2.59230084993978149299209690070711076259613037109375;0.0741333232756055948708961977899889461696147918701171875;-2.13375794863389245392681914381682872772216796875;1.6226572608943963249572561835520900785923004150390625;-0.424087116455854229446487124732811935245990753173828125;-1.3955343003322953077116608255892060697078704833984375;0.280461180516693386888249506228021346032619476318359375;-0.1145174318604867680360115400617360137403011322021484375]
      mask Display: e = 0.06;c1 = [120 150 230]/255;c2 = ([120 150 230]+0)/383;c3 = ([120 150 230]+128)/383;patch([0 1 1 0],[0 0 1 1],c1);patch([0 1 1 1-e 1-e 0+e],[0 0 1 1-e 0+e 0+e],c2);patch([0 0 1 1-e 0+e 0+e],[0 1 1 1-e 1-e 0+e],c3);plot([0 1 1 0 0],[0 0 1 1 0]);disp('weights');
  "IW{2,1}(97,:)'" : Constant  Value=[-0.3451013264426574522758528473787009716033935546875;0.660949337027847860781548661179840564727783203125;2.040444200637787641738896127208136022090911865234375;-0.64417905793472340914007645551464520394802093505859375;-2.496098599504593895659354529925622045993804931640625;1.360397222918155790694072493351995944976806640625;0.3233144786560526728891318271053023636341094970703125;0.2082367773194217785981408042061957530677318572998046875;-0.6244113070238677121182035989477299153804779052734375;0.7746133584127996574153485198621638119220733642578125]
      mask Display: e = 0.06;c1 = [120 150 230]/255;c2 = ([120 150 230]+0)/383;c3 = ([120 150 230]+128)/383;patch([0 1 1 0],[0 0 1 1],c1);patch([0 1 1 1-e 1-e 0+e],[0 0 1 1-e 0+e 0+e],c2);patch([0 0 1 1-e 0+e 0+e],[0 1 1 1-e 1-e 0+e],c3);plot([0 1 1 0 0],[0 0 1 1 0]);disp('weights');
  "IW{2,1}(98,:)'" : Constant  Value=[-0.29206332519817912451998154210741631686687469482421875;0.65744433169371097047672947155660949647426605224609375;1.9826005662397074846836630968027748167514801025390625;-0.355710703540655648335899741141474805772304534912109375;-2.215377212138320839329708178411237895488739013671875;1.2864767494380353607397182713611982762813568115234375;0.058183591502243094117918786878362880088388919830322265625;-0.34248155399259194719974175313836894929409027099609375;-1.06127678688388105143758366466499865055084228515625;0.12332252953084808788641879573333426378667354583740234375]
      mask Display: e = 0.06;c1 = [120 150 230]/255;c2 = ([120 150 230]+0)/383;c3 = ([120 150 230]+128)/383;patch([0 1 1 0],[0 0 1 1],c1);patch([0 1 1 1-e 1-e 0+e],[0 0 1 1-e 0+e 0+e],c2);patch([0 0 1 1-e 0+e 0+e],[0 1 1 1-e 1-e 0+e],c3);plot([0 1 1 0 0],[0 0 1 1 0]);disp('weights');
  "IW{2,1}(99,:)'" : Constant  Value=[-0.48545396614517299926916393815190531313419342041015625;0.68278508633127066307366703767911531031131744384765625;2.29394745233972940923194983042776584625244140625;-0.2778339498886956970835626634652726352214813232421875;-1.65508146184715787541108511504717171192169189453125;1.4802637353369034745043109069229103624820709228515625;-0.044466910029728391740011517185848788358271121978759765625;-0.01370227842365283332792813553169253282248973846435546875;-0.859303904747432678590257637551985681056976318359375;0.92080011412219864297412641462869942188262939453125]
      mask Display: e = 0.06;c1 = [120 150 230]/255;c2 = ([120 150 230]+0)/383;c3 = ([120 150 230]+128)/383;patch([0 1 1 0],[0 0 1 1],c1);patch([0 1 1 1-e 1-e 0+e],[0 0 1 1-e 0+e 0+e],c2);patch([0 0 1 1-e 0+e 0+e],[0 1 1 1-e 1-e 0+e],c3);plot([0 1 1 0 0],[0 0 1 1 0]);disp('weights');
  Mux : Mux  Inputs=100
      mask Display: e = 0.06;c1 = [120 150 230]/255;c2 = ([120 150 230]+0)/383;c3 = ([120 150 230]+128)/383;patch([0 1 1 0],[0 0 1 1],c1);patch([0 1 1 1-e 1-e 0+e],[0 0 1 1-e 0+e 0+e],c2);patch([0 0 1 1-e 0+e 0+e],[0 1 1 1-e 1-e 0+e],c3);plot([0 1 1 0 0],[0 0 1 1 0]);disp('Mux');
  dotprod{1..100} (100 alike) : neural/Weight Functions/dotprod
  "lz{2,1}" : Outport
      mask Display: e = 0.06;c1 = [120 230 180]/255;c2 = ([120 230 180]+0)/(256+128);c3 = ([120 230 180]+128)/(256+128);patch([0 1 1 0],[0 0 1 1],c1);patch([0 1 1 1-e 1-e 0+e],[0 0 1 1-e 0+e 0+e],c2);patch([0 0 1 1-e 0+e 0+e],[0 1 1 1-e 1-e 0+e],c3);plot([0 1 1 0 0],[0 0 1 1 0]);
  wires:
  "IW{2,1}(1,:)'"/1 -> dotprod1/1
  "ad{2,1}"/1 -> dotprod1/2, dotprod2/2, dotprod3/2, dotprod4/2, dotprod5/2, dotprod6/2, dotprod7/2, dotprod8/2, dotprod9/2, dotprod10/2, dotprod11/2, dotprod12/2, dotprod13/2, dotprod14/2, dotprod15/2, dotprod16/2, dotprod17/2, dotprod18/2, dotprod19/2, dotprod20/2, dotprod21/2, dotprod22/2, dotprod23/2, dotprod24/2, dotprod25/2, dotprod26/2, dotprod27/2, dotprod28/2, dotprod29/2, dotprod30/2, dotprod31/2, dotprod32/2, dotprod33/2, dotprod34/2, dotprod35/2, dotprod36/2, dotprod37/2, dotprod38/2, dotprod39/2, dotprod40/2, dotprod41/2, dotprod42/2, dotprod43/2, dotprod44/2, dotprod45/2, dotprod46/2, dotprod47/2, dotprod48/2, dotprod49/2, dotprod50/2, dotprod51/2, dotprod52/2, dotprod53/2, dotprod54/2, dotprod55/2, dotprod56/2, dotprod57/2, dotprod58/2, dotprod59/2, dotprod60/2, dotprod61/2, dotprod62/2, dotprod63/2, dotprod64/2, dotprod65/2, dotprod66/2, dotprod67/2, dotprod68/2, dotprod69/2, dotprod70/2, dotprod71/2, dotprod72/2, dotprod73/2, dotprod74/2, dotprod75/2, dotprod76/2, dotprod77/2, dotprod78/2, dotprod79/2, dotprod80/2, dotprod81/2, dotprod82/2, dotprod83/2, dotprod84/2, dotprod85/2, dotprod86/2, dotprod87/2, dotprod88/2, dotprod89/2, dotprod90/2, dotprod91/2, dotprod92/2, dotprod93/2, dotprod94/2, dotprod95/2, dotprod96/2, dotprod97/2, dotprod98/2, dotprod99/2, dotprod100/2
  dotprod1/1 -> Mux/1
  "IW{2,1}(2,:)'"/1 -> dotprod2/1
  dotprod2/1 -> Mux/2
  "IW{2,1}(3,:)'"/1 -> dotprod3/1
  dotprod3/1 -> Mux/3
  "IW{2,1}(4,:)'"/1 -> dotprod4/1
  dotprod4/1 -> Mux/4
  "IW{2,1}(5,:)'"/1 -> dotprod5/1
  dotprod5/1 -> Mux/5
  "IW{2,1}(6,:)'"/1 -> dotprod6/1
  dotprod6/1 -> Mux/6
  "IW{2,1}(7,:)'"/1 -> dotprod7/1
  dotprod7/1 -> Mux/7
  "IW{2,1}(8,:)'"/1 -> dotprod8/1
  dotprod8/1 -> Mux/8
  "IW{2,1}(9,:)'"/1 -> dotprod9/1
  dotprod9/1 -> Mux/9
  "IW{2,1}(10,:)'"/1 -> dotprod10/1
  dotprod10/1 -> Mux/10
  "IW{2,1}(11,:)'"/1 -> dotprod11/1
  dotprod11/1 -> Mux/11
  "IW{2,1}(12,:)'"/1 -> dotprod12/1
  dotprod12/1 -> Mux/12
  "IW{2,1}(13,:)'"/1 -> dotprod13/1
  dotprod13/1 -> Mux/13
  "IW{2,1}(14,:)'"/1 -> dotprod14/1
  dotprod14/1 -> Mux/14
  "IW{2,1}(15,:)'"/1 -> dotprod15/1
  dotprod15/1 -> Mux/15
  "IW{2,1}(16,:)'"/1 -> dotprod16/1
  dotprod16/1 -> Mux/16
  "IW{2,1}(17,:)'"/1 -> dotprod17/1
  dotprod17/1 -> Mux/17
  "IW{2,1}(18,:)'"/1 -> dotprod18/1
  dotprod18/1 -> Mux/18
  "IW{2,1}(19,:)'"/1 -> dotprod19/1
  dotprod19/1 -> Mux/19
  "IW{2,1}(20,:)'"/1 -> dotprod20/1
  dotprod20/1 -> Mux/20
  "IW{2,1}(21,:)'"/1 -> dotprod21/1
  dotprod21/1 -> Mux/21
  "IW{2,1}(22,:)'"/1 -> dotprod22/1
  dotprod22/1 -> Mux/22
  "IW{2,1}(23,:)'"/1 -> dotprod23/1
  dotprod23/1 -> Mux/23
  "IW{2,1}(24,:)'"/1 -> dotprod24/1
  dotprod24/1 -> Mux/24
  "IW{2,1}(25,:)'"/1 -> dotprod25/1
  dotprod25/1 -> Mux/25
  "IW{2,1}(26,:)'"/1 -> dotprod26/1
  dotprod26/1 -> Mux/26
  "IW{2,1}(27,:)'"/1 -> dotprod27/1
  dotprod27/1 -> Mux/27
  "IW{2,1}(28,:)'"/1 -> dotprod28/1
  dotprod28/1 -> Mux/28
  "IW{2,1}(29,:)'"/1 -> dotprod29/1
  dotprod29/1 -> Mux/29
  "IW{2,1}(30,:)'"/1 -> dotprod30/1
  dotprod30/1 -> Mux/30
  "IW{2,1}(31,:)'"/1 -> dotprod31/1
  dotprod31/1 -> Mux/31
  "IW{2,1}(32,:)'"/1 -> dotprod32/1
  dotprod32/1 -> Mux/32
  "IW{2,1}(33,:)'"/1 -> dotprod33/1
  dotprod33/1 -> Mux/33
  "IW{2,1}(34,:)'"/1 -> dotprod34/1
  dotprod34/1 -> Mux/34
  "IW{2,1}(35,:)'"/1 -> dotprod35/1
  dotprod35/1 -> Mux/35
  "IW{2,1}(36,:)'"/1 -> dotprod36/1
  dotprod36/1 -> Mux/36
  "IW{2,1}(37,:)'"/1 -> dotprod37/1
  dotprod37/1 -> Mux/37
  "IW{2,1}(38,:)'"/1 -> dotprod38/1
  dotprod38/1 -> Mux/38
  "IW{2,1}(39,:)'"/1 -> dotprod39/1
  dotprod39/1 -> Mux/39
  "IW{2,1}(40,:)'"/1 -> dotprod40/1
  dotprod40/1 -> Mux/40
  "IW{2,1}(41,:)'"/1 -> dotprod41/1
  dotprod41/1 -> Mux/41
  "IW{2,1}(42,:)'"/1 -> dotprod42/1
  dotprod42/1 -> Mux/42
  "IW{2,1}(43,:)'"/1 -> dotprod43/1
  dotprod43/1 -> Mux/43
  "IW{2,1}(44,:)'"/1 -> dotprod44/1
  dotprod44/1 -> Mux/44
  "IW{2,1}(45,:)'"/1 -> dotprod45/1
  dotprod45/1 -> Mux/45
  "IW{2,1}(46,:)'"/1 -> dotprod46/1
  dotprod46/1 -> Mux/46
  "IW{2,1}(47,:)'"/1 -> dotprod47/1
  dotprod47/1 -> Mux/47
  "IW{2,1}(48,:)'"/1 -> dotprod48/1
  dotprod48/1 -> Mux/48
  "IW{2,1}(49,:)'"/1 -> dotprod49/1
  dotprod49/1 -> Mux/49
  "IW{2,1}(50,:)'"/1 -> dotprod50/1
  dotprod50/1 -> Mux/50
  "IW{2,1}(51,:)'"/1 -> dotprod51/1
  dotprod51/1 -> Mux/51
  "IW{2,1}(52,:)'"/1 -> dotprod52/1
  dotprod52/1 -> Mux/52
  "IW{2,1}(53,:)'"/1 -> dotprod53/1
  dotprod53/1 -> Mux/53
  "IW{2,1}(54,:)'"/1 -> dotprod54/1
  dotprod54/1 -> Mux/54
  "IW{2,1}(55,:)'"/1 -> dotprod55/1
  dotprod55/1 -> Mux/55
  "IW{2,1}(56,:)'"/1 -> dotprod56/1
  dotprod56/1 -> Mux/56
  "IW{2,1}(57,:)'"/1 -> dotprod57/1
  dotprod57/1 -> Mux/57
  "IW{2,1}(58,:)'"/1 -> dotprod58/1
  dotprod58/1 -> Mux/58
  "IW{2,1}(59,:)'"/1 -> dotprod59/1
  dotprod59/1 -> Mux/59
  "IW{2,1}(60,:)'"/1 -> dotprod60/1
  dotprod60/1 -> Mux/60
  "IW{2,1}(61,:)'"/1 -> dotprod61/1
  dotprod61/1 -> Mux/61
  "IW{2,1}(62,:)'"/1 -> dotprod62/1
  dotprod62/1 -> Mux/62
  "IW{2,1}(63,:)'"/1 -> dotprod63/1
  dotprod63/1 -> Mux/63
  "IW{2,1}(64,:)'"/1 -> dotprod64/1
  dotprod64/1 -> Mux/64
  "IW{2,1}(65,:)'"/1 -> dotprod65/1
  dotprod65/1 -> Mux/65
  "IW{2,1}(66,:)'"/1 -> dotprod66/1
  dotprod66/1 -> Mux/66
  "IW{2,1}(67,:)'"/1 -> dotprod67/1
  dotprod67/1 -> Mux/67
  "IW{2,1}(68,:)'"/1 -> dotprod68/1
  dotprod68/1 -> Mux/68
  "IW{2,1}(69,:)'"/1 -> dotprod69/1
  dotprod69/1 -> Mux/69
  "IW{2,1}(70,:)'"/1 -> dotprod70/1
  dotprod70/1 -> Mux/70
  "IW{2,1}(71,:)'"/1 -> dotprod71/1
  dotprod71/1 -> Mux/71
  "IW{2,1}(72,:)'"/1 -> dotprod72/1
  dotprod72/1 -> Mux/72
  "IW{2,1}(73,:)'"/1 -> dotprod73/1
  dotprod73/1 -> Mux/73
  "IW{2,1}(74,:)'"/1 -> dotprod74/1
  dotprod74/1 -> Mux/74
  "IW{2,1}(75,:)'"/1 -> dotprod75/1
  dotprod75/1 -> Mux/75
  "IW{2,1}(76,:)'"/1 -> dotprod76/1
  dotprod76/1 -> Mux/76
  "IW{2,1}(77,:)'"/1 -> dotprod77/1
  dotprod77/1 -> Mux/77
  "IW{2,1}(78,:)'"/1 -> dotprod78/1
  dotprod78/1 -> Mux/78
  "IW{2,1}(79,:)'"/1 -> dotprod79/1
  dotprod79/1 -> Mux/79
  "IW{2,1}(80,:)'"/1 -> dotprod80/1
  dotprod80/1 -> Mux/80
  "IW{2,1}(81,:)'"/1 -> dotprod81/1
  dotprod81/1 -> Mux/81
  "IW{2,1}(82,:)'"/1 -> dotprod82/1
  dotprod82/1 -> Mux/82
  "IW{2,1}(83,:)'"/1 -> dotprod83/1
  dotprod83/1 -> Mux/83
  "IW{2,1}(84,:)'"/1 -> dotprod84/1
  dotprod84/1 -> Mux/84
  "IW{2,1}(85,:)'"/1 -> dotprod85/1
  dotprod85/1 -> Mux/85
  "IW{2,1}(86,:)'"/1 -> dotprod86/1
  dotprod86/1 -> Mux/86
  "IW{2,1}(87,:)'"/1 -> dotprod87/1
  dotprod87/1 -> Mux/87
  "IW{2,1}(88,:)'"/1 -> dotprod88/1
  dotprod88/1 -> Mux/88
  "IW{2,1}(89,:)'"/1 -> dotprod89/1
  dotprod89/1 -> Mux/89
  "IW{2,1}(90,:)'"/1 -> dotprod90/1
  dotprod90/1 -> Mux/90
  "IW{2,1}(91,:)'"/1 -> dotprod91/1
  dotprod91/1 -> Mux/91
  "IW{2,1}(92,:)'"/1 -> dotprod92/1
  dotprod92/1 -> Mux/92
  "IW{2,1}(93,:)'"/1 -> dotprod93/1
  dotprod93/1 -> Mux/93
  "IW{2,1}(94,:)'"/1 -> dotprod94/1
  dotprod94/1 -> Mux/94
  "IW{2,1}(95,:)'"/1 -> dotprod95/1
  dotprod95/1 -> Mux/95
  "IW{2,1}(96,:)'"/1 -> dotprod96/1
  dotprod96/1 -> Mux/96
  "IW{2,1}(97,:)'"/1 -> dotprod97/1
  dotprod97/1 -> Mux/97
  "IW{2,1}(98,:)'"/1 -> dotprod98/1
  dotprod98/1 -> Mux/98
  "IW{2,1}(99,:)'"/1 -> dotprod99/1
  dotprod99/1 -> Mux/99
  "IW{2,1}(100,:)'"/1 -> dotprod100/1
  dotprod100/1 -> Mux/100
  Mux/1 -> "lz{2,1}"/1
